simulink library "outp"  (R2021b)
(part 5 of 7)

  VPMM_ActiveDischargeReq_flg_Inproc : FVT_lib/outp/OverrideAndLimit  SystemSampleTime=-1  VariantActivationTime=update diagram  Latency=0  AutoFrameSizeCalculation=off
      link override Signal_Limit/_maxval: Value=KOUTP_ActiveDischargeReq_flg_maxval
      link override Signal_Limit/_minval: Value=KOUTP_ActiveDischargeReq_flg_minval
      link override Signal_Override/_ovrdflg: Value=KOUTP_ActiveDischargeReq_flg_ovrdflg
      link override Signal_Override/_ovrdval: Value=KOUTP_ActiveDischargeReq_flg_ovrdval
  VPMM_CtrlDrPwrStbA2_flg_Inproc : FVT_lib/outp/OverrideAndLimit  SystemSampleTime=-1  VariantActivationTime=update diagram  Latency=0  AutoFrameSizeCalculation=off
      link override Signal_Limit/_maxval: Value=KOUTP_CtrlDrPwrStbA2_flg_maxval
      link override Signal_Limit/_minval: Value=KOUTP_CtrlDrPwrStbA2_flg_minval
      link override Signal_Override/_ovrdflg: Value=KOUTP_CtrlDrPwrStbA2_flg_ovrdflg
      link override Signal_Override/_ovrdval: Value=KOUTP_CtrlDrPwrStbA2_flg_ovrdval
  VPMM_CtrlFrBMSCCUCIR_flg_Inproc : FVT_lib/outp/OverrideAndLimit  SystemSampleTime=-1  VariantActivationTime=update diagram  Latency=0  AutoFrameSizeCalculation=off
      link override Signal_Limit/_maxval: Value=KOUTP_CtrlFrBMSCCUCIR_flg_maxval
      link override Signal_Limit/_minval: Value=KOUTP_CtrlFrBMSCCUCIR_flg_minval
      link override Signal_Override/_ovrdflg: Value=KOUTP_CtrlFrBMSCCUCIR_flg_ovrdflg
      link override Signal_Override/_ovrdval: Value=KOUTP_CtrlFrBMSCCUCIR_flg_ovrdval
  VPMM_CtrlFrEDUINVERTER_flg_Inproc : FVT_lib/outp/OverrideAndLimit  SystemSampleTime=-1  VariantActivationTime=update diagram  Latency=0  AutoFrameSizeCalculation=off
      link override Signal_Limit/_maxval: Value=KOUTP_CtrlFrEDUINVERTER_flg_maxval
      link override Signal_Limit/_minval: Value=KOUTP_CtrlFrEDUINVERTER_flg_minval
      link override Signal_Override/_ovrdflg: Value=KOUTP_CtrlFrEDUINVERTER_flg_ovrdflg
      link override Signal_Override/_ovrdval: Value=KOUTP_CtrlFrEDUINVERTER_flg_ovrdval
  VPMM_CtrlFrPwrStbA1P_flg_Inproc : FVT_lib/outp/OverrideAndLimit  SystemSampleTime=-1  VariantActivationTime=update diagram  Latency=0  AutoFrameSizeCalculation=off
      link override Signal_Limit/_maxval: Value=KOUTP_CtrlFrPwrStbA1P_flg_maxval
      link override Signal_Limit/_minval: Value=KOUTP_CtrlFrPwrStbA1P_flg_minval
      link override Signal_Override/_ovrdflg: Value=KOUTP_CtrlFrPwrStbA1P_flg_ovrdflg
      link override Signal_Override/_ovrdval: Value=KOUTP_CtrlFrPwrStbA1P_flg_ovrdval
  VPMM_CtrlFrRC1_flg_Inproc : FVT_lib/outp/OverrideAndLimit  SystemSampleTime=-1  VariantActivationTime=update diagram  Latency=0  AutoFrameSizeCalculation=off
      link override Signal_Limit/_maxval: Value=KOUTP_CtrlFrRC1_flg_maxval
      link override Signal_Limit/_minval: Value=KOUTP_CtrlFrRC1_flg_minval
      link override Signal_Override/_ovrdflg: Value=KOUTP_CtrlFrRC1_flg_ovrdflg
      link override Signal_Override/_ovrdval: Value=KOUTP_CtrlFrRC1_flg_ovrdval
  VPMM_DCDCEnDem_enum_Inproc : FVT_lib/outp/OverrideAndLimit  SystemSampleTime=-1  VariantActivationTime=update diagram  Latency=0  AutoFrameSizeCalculation=off
      link override Signal_Limit/_maxval: Value=KOUTP_DCDCEnDem_enum_maxval
      link override Signal_Limit/_minval: Value=KOUTP_DCDCEnDem_enum_minval
      link override Signal_Override/_ovrdflg: Value=KOUTP_DCDCEnDem_enum_ovrdflg
      link override Signal_Override/_ovrdval: Value=KOUTP_DCDCEnDem_enum_ovrdval
  VPMM_DCDCEnaReq_flg_Inproc : FVT_lib/outp/OverrideAndLimit  SystemSampleTime=-1  VariantActivationTime=update diagram  Latency=0  AutoFrameSizeCalculation=off
      link override Signal_Limit/_maxval: Value=KOUTP_DCDCEnaReq_flg_maxval
      link override Signal_Limit/_minval: Value=KOUTP_DCDCEnaReq_flg_minval
      link override Signal_Override/_ovrdflg: Value=KOUTP_DCDCEnaReq_flg_ovrdflg
      link override Signal_Override/_ovrdval: Value=KOUTP_DCDCEnaReq_flg_ovrdval
  VPMM_DCDCRlyDem_enum_Inproc : FVT_lib/outp/OverrideAndLimit  SystemSampleTime=-1  VariantActivationTime=update diagram  Latency=0  AutoFrameSizeCalculation=off
      link override Signal_Limit/_maxval: Value=KOUTP_DCDCRlyDem_enum_maxval
      link override Signal_Limit/_minval: Value=KOUTP_DCDCRlyDem_enum_minval
      link override Signal_Override/_ovrdflg: Value=KOUTP_DCDCRlyDem_enum_ovrdflg
      link override Signal_Override/_ovrdval: Value=KOUTP_DCDCRlyDem_enum_ovrdval
  VPMM_DCDCVoltSetpoint_V_Inproc : FVT_lib/outp/OverrideAndLimit  SystemSampleTime=-1  VariantActivationTime=update diagram  Latency=0  AutoFrameSizeCalculation=off
      link override Signal_Limit/_maxval: Value=KOUTP_DCDCVoltSetpoint_V_maxval
      link override Signal_Limit/_minval: Value=KOUTP_DCDCVoltSetpoint_V_minval
      link override Signal_Override/_ovrdflg: Value=KOUTP_DCDCVoltSetpoint_V_ovrdflg
      link override Signal_Override/_ovrdval: Value=KOUTP_DCDCVoltSetpoint_V_ovrdval
  VPMM_DrSeatSta_enum_Inproc : FVT_lib/outp/OverrideAndLimit  SystemSampleTime=-1  VariantActivationTime=update diagram  Latency=0  AutoFrameSizeCalculation=off
      link override Signal_Limit/_maxval: Value=KOUTP_DrSeatSta_enum_maxval
      link override Signal_Limit/_minval: Value=KOUTP_DrSeatSta_enum_minval
      link override Signal_Override/_ovrdflg: Value=KOUTP_DrSeatSta_enum_ovrdflg
      link override Signal_Override/_ovrdval: Value=KOUTP_DrSeatSta_enum_ovrdval
  VPMM_DrivetrainSelect_enum_Inproc : FVT_lib/outp/OverrideAndLimit  SystemSampleTime=-1  VariantActivationTime=update diagram  Latency=0  AutoFrameSizeCalculation=off
      link override Signal_Limit/_maxval: Value=KOUTP_DrivetrainSelect_enum_maxval
      link override Signal_Limit/_minval: Value=KOUTP_DrivetrainSelect_enum_minval
      link override Signal_Override/_ovrdflg: Value=KOUTP_DrivetrainSelect_enum_ovrdflg
      link override Signal_Override/_ovrdval: Value=KOUTP_DrivetrainSelect_enum_ovrdval
  VPMM_EACRlyDem_enum_Inproc : FVT_lib/outp/OverrideAndLimit  SystemSampleTime=-1  VariantActivationTime=update diagram  Latency=0  AutoFrameSizeCalculation=off
      link override Signal_Limit/_maxval: Value=KOUTP_EACRlyDem_enum_maxval
      link override Signal_Limit/_minval: Value=KOUTP_EACRlyDem_enum_minval
      link override Signal_Override/_ovrdflg: Value=KOUTP_EACRlyDem_enum_ovrdflg
      link override Signal_Override/_ovrdval: Value=KOUTP_EACRlyDem_enum_ovrdval
  VPMM_EHPSRlyDem_enum_Inproc : FVT_lib/outp/OverrideAndLimit  SystemSampleTime=-1  VariantActivationTime=update diagram  Latency=0  AutoFrameSizeCalculation=off
      link override Signal_Limit/_maxval: Value=KOUTP_EHPSRlyDem_enum_maxval
      link override Signal_Limit/_minval: Value=KOUTP_EHPSRlyDem_enum_minval
      link override Signal_Override/_ovrdflg: Value=KOUTP_EHPSRlyDem_enum_ovrdflg
      link override Signal_Override/_ovrdval: Value=KOUTP_EHPSRlyDem_enum_ovrdval
  VPMM_EvccAplusPwrUpReq_flg_Inproc : FVT_lib/outp/OverrideAndLimit  SystemSampleTime=-1  VariantActivationTime=update diagram  Latency=0  AutoFrameSizeCalculation=off
      link override Signal_Limit/_maxval: Value=KOUTP_EvccAplusPwrUpReq_flg_maxval
      link override Signal_Limit/_minval: Value=KOUTP_EvccAplusPwrUpReq_flg_minval
      link override Signal_Override/_ovrdflg: Value=KOUTP_EvccAplusPwrUpReq_flg_ovrdflg
      link override Signal_Override/_ovrdval: Value=KOUTP_EvccAplusPwrUpReq_flg_ovrdval
  VPMM_FDADC12VDetAvg_mV_Inproc : FVT_lib/outp/OverrideAndLimit  SystemSampleTime=-1  VariantActivationTime=update diagram  Latency=0  AutoFrameSizeCalculation=off
      link override Signal_Limit/_maxval: Value=KOUTP_FDADC12VDetAvg_mV_maxval
      link override Signal_Limit/_minval: Value=KOUTP_FDADC12VDetAvg_mV_minval
      link override Signal_Override/_ovrdflg: Value=KOUTP_FDADC12VDetAvg_mV_ovrdflg
      link override Signal_Override/_ovrdval: Value=KOUTP_FDADC12VDetAvg_mV_ovrdval
  VPMM_FrMCUEnaReq_flg_Inproc : FVT_lib/outp/OverrideAndLimit  SystemSampleTime=-1  VariantActivationTime=update diagram  Latency=0  AutoFrameSizeCalculation=off
      link override Signal_Limit/_maxval: Value=KOUTP_FrMCUEnaReq_flg_maxval
      link override Signal_Limit/_minval: Value=KOUTP_FrMCUEnaReq_flg_minval
      link override Signal_Override/_ovrdflg: Value=KOUTP_FrMCUEnaReq_flg_ovrdflg
      link override Signal_Override/_ovrdval: Value=KOUTP_FrMCUEnaReq_flg_ovrdval
  VPMM_HVBatCnctReq_flg_Inproc : FVT_lib/outp/OverrideAndLimit  SystemSampleTime=-1  VariantActivationTime=update diagram  Latency=0  AutoFrameSizeCalculation=off
      link override Signal_Limit/_maxval: Value=KOUTP_HVBatCnctReq_flg_maxval
      link override Signal_Limit/_minval: Value=KOUTP_HVBatCnctReq_flg_minval
      link override Signal_Override/_ovrdflg: Value=KOUTP_HVBatCnctReq_flg_ovrdflg
      link override Signal_Override/_ovrdval: Value=KOUTP_HVBatCnctReq_flg_ovrdval
  VPMM_HVPwrSta_flg_Inproc : FVT_lib/outp/OverrideAndLimit  SystemSampleTime=-1  VariantActivationTime=update diagram  Latency=0  AutoFrameSizeCalculation=off
      link override Signal_Limit/_maxval: Value=KOUTP_HVPwrSta_flg_maxval
      link override Signal_Limit/_minval: Value=KOUTP_HVPwrSta_flg_minval
      link override Signal_Override/_ovrdflg: Value=KOUTP_HVPwrSta_flg_ovrdflg
      link override Signal_Override/_ovrdval: Value=KOUTP_HVPwrSta_flg_ovrdval
  VPMM_HVSysReadyToCharge_enum_Inproc : FVT_lib/outp/OverrideAndLimit  SystemSampleTime=-1  VariantActivationTime=update diagram  Latency=0  AutoFrameSizeCalculation=off
      link override Signal_Limit/_maxval: Value=KOUTP_HVSysReadyToCharge_enum_maxval
      link override Signal_Limit/_minval: Value=KOUTP_HVSysReadyToCharge_enum_minval
      link override Signal_Override/_ovrdflg: Value=KOUTP_HVSysReadyToCharge_enum_ovrdflg
      link override Signal_Override/_ovrdval: Value=KOUTP_HVSysReadyToCharge_enum_ovrdval
  VPMM_HWResetSta_enum_Inproc : FVT_lib/outp/OverrideAndLimit  SystemSampleTime=-1  VariantActivationTime=update diagram  Latency=0  AutoFrameSizeCalculation=off
      link override Signal_Limit/_maxval: Value=KOUTP_HWResetSta_enum_maxval
      link override Signal_Limit/_minval: Value=KOUTP_HWResetSta_enum_minval
      link override Signal_Override/_ovrdflg: Value=KOUTP_HWResetSta_enum_ovrdflg
      link override Signal_Override/_ovrdval: Value=KOUTP_HWResetSta_enum_ovrdval
  VPMM_IVIPwrStaONTOPopT_s_Inproc : FVT_lib/outp/OverrideAndLimit  SystemSampleTime=-1  VariantActivationTime=update diagram  Latency=0  AutoFrameSizeCalculation=off
      link override Signal_Limit/_maxval: Value=KOUTP_IVIPwrStaONTOPopT_s_maxval
      link override Signal_Limit/_minval: Value=KOUTP_IVIPwrStaONTOPopT_s_minval
      link override Signal_Override/_ovrdflg: Value=KOUTP_IVIPwrStaONTOPopT_s_ovrdflg
      link override Signal_Override/_ovrdval: Value=KOUTP_IVIPwrStaONTOPopT_s_ovrdval
  VPMM_LVBattChrgTimeCnt_s_Inproc : FVT_lib/outp/OverrideAndLimit  SystemSampleTime=-1  VariantActivationTime=update diagram  Latency=0  AutoFrameSizeCalculation=off
      link override Signal_Limit/_maxval: Value=KOUTP_LVBattChrgTimeCnt_s_maxval
      link override Signal_Limit/_minval: Value=KOUTP_LVBattChrgTimeCnt_s_minval
      link override Signal_Override/_ovrdflg: Value=KOUTP_LVBattChrgTimeCnt_s_ovrdflg
      link override Signal_Override/_ovrdval: Value=KOUTP_LVBattChrgTimeCnt_s_ovrdval
  VPMM_LVChrgHoldTtimer_s_Inproc : FVT_lib/outp/OverrideAndLimit  SystemSampleTime=-1  VariantActivationTime=update diagram  Latency=0  AutoFrameSizeCalculation=off
      link override Signal_Limit/_maxval: Value=KOUTP_LVChrgHoldTtimer_s_maxval
      link override Signal_Limit/_minval: Value=KOUTP_LVChrgHoldTtimer_s_minval
      link override Signal_Override/_ovrdflg: Value=KOUTP_LVChrgHoldTtimer_s_ovrdflg
      link override Signal_Override/_ovrdval: Value=KOUTP_LVChrgHoldTtimer_s_ovrdval
  VPMM_LVPwrSta_flg_Inproc : FVT_lib/outp/OverrideAndLimit  SystemSampleTime=-1  VariantActivationTime=update diagram  Latency=0  AutoFrameSizeCalculation=off
      link override Signal_Limit/_maxval: Value=KOUTP_LVPwrSta_flg_maxval
      link override Signal_Limit/_minval: Value=KOUTP_LVPwrSta_flg_minval
      link override Signal_Override/_ovrdflg: Value=KOUTP_LVPwrSta_flg_ovrdflg
      link override Signal_Override/_ovrdval: Value=KOUTP_LVPwrSta_flg_ovrdval
  VPMM_LVSilentChrgLv_enum_Inproc : FVT_lib/outp/OverrideAndLimit  SystemSampleTime=-1  VariantActivationTime=update diagram  Latency=0  AutoFrameSizeCalculation=off
      link override Signal_Limit/_maxval: Value=KOUTP_LVSilentChrgLv_enum_maxval
      link override Signal_Limit/_minval: Value=KOUTP_LVSilentChrgLv_enum_minval
      link override Signal_Override/_ovrdflg: Value=KOUTP_LVSilentChrgLv_enum_ovrdflg
      link override Signal_Override/_ovrdval: Value=KOUTP_LVSilentChrgLv_enum_ovrdval
  VPMM_LVSilentChrgReq_flg_Inproc : FVT_lib/outp/OverrideAndLimit  SystemSampleTime=-1  VariantActivationTime=update diagram  Latency=0  AutoFrameSizeCalculation=off
      link override Signal_Limit/_maxval: Value=KOUTP_LVSilentChrgReq_flg_maxval
      link override Signal_Limit/_minval: Value=KOUTP_LVSilentChrgReq_flg_minval
      link override Signal_Override/_ovrdflg: Value=KOUTP_LVSilentChrgReq_flg_ovrdflg
      link override Signal_Override/_ovrdval: Value=KOUTP_LVSilentChrgReq_flg_ovrdval
  VPMM_LVSilentChrgSta_enum_Inproc : FVT_lib/outp/OverrideAndLimit  SystemSampleTime=-1  VariantActivationTime=update diagram  Latency=0  AutoFrameSizeCalculation=off
      link override Signal_Limit/_maxval: Value=KOUTP_LVSilentChrgSta_enum_maxval
      link override Signal_Limit/_minval: Value=KOUTP_LVSilentChrgSta_enum_minval
      link override Signal_Override/_ovrdflg: Value=KOUTP_LVSilentChrgSta_enum_ovrdflg
      link override Signal_Override/_ovrdval: Value=KOUTP_LVSilentChrgSta_enum_ovrdval
  VPMM_LVSysErrPwrOutErr_flg_Inproc : FVT_lib/outp/OverrideAndLimit  SystemSampleTime=-1  VariantActivationTime=update diagram  Latency=0  AutoFrameSizeCalculation=off
      link override Signal_Limit/_maxval: Value=KOUTP_LVSysErrPwrOutErr_flg_maxval
      link override Signal_Limit/_minval: Value=KOUTP_LVSysErrPwrOutErr_flg_minval
      link override Signal_Override/_ovrdflg: Value=KOUTP_LVSysErrPwrOutErr_flg_ovrdflg
      link override Signal_Override/_ovrdval: Value=KOUTP_LVSysErrPwrOutErr_flg_ovrdval
  VPMM_LowSOCWarn_enum_Inproc : FVT_lib/outp/OverrideAndLimit  SystemSampleTime=-1  VariantActivationTime=update diagram  Latency=0  AutoFrameSizeCalculation=off
      link override Signal_Limit/_maxval: Value=KOUTP_LowSOCWarn_enum_maxval
      link override Signal_Limit/_minval: Value=KOUTP_LowSOCWarn_enum_minval
      link override Signal_Override/_ovrdflg: Value=KOUTP_LowSOCWarn_enum_ovrdflg
      link override Signal_Override/_ovrdval: Value=KOUTP_LowSOCWarn_enum_ovrdval
  VPMM_PMMAllowECUSleep_flg_Inproc : FVT_lib/outp/OverrideAndLimit  SystemSampleTime=-1  VariantActivationTime=update diagram  Latency=0  AutoFrameSizeCalculation=off
      link override Signal_Limit/_maxval: Value=KOUTP_PMMAllowECUSleep_flg_maxval
      link override Signal_Limit/_minval: Value=KOUTP_PMMAllowECUSleep_flg_minval
      link override Signal_Override/_ovrdflg: Value=KOUTP_PMMAllowECUSleep_flg_ovrdflg
      link override Signal_Override/_ovrdval: Value=KOUTP_PMMAllowECUSleep_flg_ovrdval
  VPMM_PowerDownFault_enum_Inproc : FVT_lib/outp/OverrideAndLimit  SystemSampleTime=-1  VariantActivationTime=update diagram  Latency=0  AutoFrameSizeCalculation=off
      link override Signal_Limit/_maxval: Value=KOUTP_PowerDownFault_enum_maxval
      link override Signal_Limit/_minval: Value=KOUTP_PowerDownFault_enum_minval
      link override Signal_Override/_ovrdflg: Value=KOUTP_PowerDownFault_enum_ovrdflg
      link override Signal_Override/_ovrdval: Value=KOUTP_PowerDownFault_enum_ovrdval
  VPMM_PowerDownState_enum_Inproc : FVT_lib/outp/OverrideAndLimit  SystemSampleTime=-1  VariantActivationTime=update diagram  Latency=0  AutoFrameSizeCalculation=off
      link override Signal_Limit/_maxval: Value=KOUTP_PowerDownState_enum_maxval
      link override Signal_Limit/_minval: Value=KOUTP_PowerDownState_enum_minval
      link override Signal_Override/_ovrdflg: Value=KOUTP_PowerDownState_enum_ovrdflg
      link override Signal_Override/_ovrdval: Value=KOUTP_PowerDownState_enum_ovrdval
  VPMM_PowerSta_enum_Inproc : FVT_lib/outp/OverrideAndLimit  SystemSampleTime=-1  VariantActivationTime=update diagram  Latency=0  AutoFrameSizeCalculation=off
      link override Signal_Limit/_maxval: Value=KOUTP_PowerSta_enum_maxval
      link override Signal_Limit/_minval: Value=KOUTP_PowerSta_enum_minval
      link override Signal_Override/_ovrdflg: Value=KOUTP_PowerSta_enum_ovrdflg
      link override Signal_Override/_ovrdval: Value=KOUTP_PowerSta_enum_ovrdval
  VPMM_PowerUpFault_enum_Inproc : FVT_lib/outp/OverrideAndLimit  SystemSampleTime=-1  VariantActivationTime=update diagram  Latency=0  AutoFrameSizeCalculation=off
      link override Signal_Limit/_maxval: Value=KOUTP_PowerUpFault_enum_maxval
      link override Signal_Limit/_minval: Value=KOUTP_PowerUpFault_enum_minval
      link override Signal_Override/_ovrdflg: Value=KOUTP_PowerUpFault_enum_ovrdflg
      link override Signal_Override/_ovrdval: Value=KOUTP_PowerUpFault_enum_ovrdval
  VPMM_PowerUpState_enum_Inproc : FVT_lib/outp/OverrideAndLimit  SystemSampleTime=-1  VariantActivationTime=update diagram  Latency=0  AutoFrameSizeCalculation=off
      link override Signal_Limit/_maxval: Value=KOUTP_PowerUpState_enum_maxval
      link override Signal_Limit/_minval: Value=KOUTP_PowerUpState_enum_minval
      link override Signal_Override/_ovrdflg: Value=KOUTP_PowerUpState_enum_ovrdflg
      link override Signal_Override/_ovrdval: Value=KOUTP_PowerUpState_enum_ovrdval
  VPMM_PwrDownReq_enum_Inproc : FVT_lib/outp/OverrideAndLimit  SystemSampleTime=-1  VariantActivationTime=update diagram  Latency=0  AutoFrameSizeCalculation=off
      link override Signal_Limit/_maxval: Value=KOUTP_PwrDownReq_enum_maxval
      link override Signal_Limit/_minval: Value=KOUTP_PwrDownReq_enum_minval
      link override Signal_Override/_ovrdflg: Value=KOUTP_PwrDownReq_enum_ovrdflg
      link override Signal_Override/_ovrdval: Value=KOUTP_PwrDownReq_enum_ovrdval
  VPMM_PwrStaConstraint_enum_Inproc : FVT_lib/outp/OverrideAndLimit  SystemSampleTime=-1  VariantActivationTime=update diagram  Latency=0  AutoFrameSizeCalculation=off
      link override Signal_Limit/_maxval: Value=KOUTP_PwrStaConstraint_enum_maxval
      link override Signal_Limit/_minval: Value=KOUTP_PwrStaConstraint_enum_minval
      link override Signal_Override/_ovrdflg: Value=KOUTP_PwrStaConstraint_enum_ovrdflg
      link override Signal_Override/_ovrdval: Value=KOUTP_PwrStaConstraint_enum_ovrdval
  VPMM_PwrStaONTOPopReq_flg_Inproc : FVT_lib/outp/OverrideAndLimit  SystemSampleTime=-1  VariantActivationTime=update diagram  Latency=0  AutoFrameSizeCalculation=off
      link override Signal_Limit/_maxval: Value=KOUTP_PwrStaONTOPopReq_flg_maxval
      link override Signal_Limit/_minval: Value=KOUTP_PwrStaONTOPopReq_flg_minval
      link override Signal_Override/_ovrdflg: Value=KOUTP_PwrStaONTOPopReq_flg_ovrdflg
      link override Signal_Override/_ovrdval: Value=KOUTP_PwrStaONTOPopReq_flg_ovrdval
  VPMM_PwrStaSelect_enum_Inproc : FVT_lib/outp/OverrideAndLimit  SystemSampleTime=-1  VariantActivationTime=update diagram  Latency=0  AutoFrameSizeCalculation=off
      link override Signal_Limit/_maxval: Value=KOUTP_PwrStaSelect_enum_maxval
      link override Signal_Limit/_minval: Value=KOUTP_PwrStaSelect_enum_minval
      link override Signal_Override/_ovrdflg: Value=KOUTP_PwrStaSelect_enum_ovrdflg
      link override Signal_Override/_ovrdval: Value=KOUTP_PwrStaSelect_enum_ovrdval
  VPMM_PwrStaTOSta_enum_Inproc : FVT_lib/outp/OverrideAndLimit  SystemSampleTime=-1  VariantActivationTime=update diagram  Latency=0  AutoFrameSizeCalculation=off
      link override Signal_Limit/_maxval: Value=KOUTP_PwrStaTOSta_enum_maxval
      link override Signal_Limit/_minval: Value=KOUTP_PwrStaTOSta_enum_minval
      link override Signal_Override/_ovrdflg: Value=KOUTP_PwrStaTOSta_enum_ovrdflg
      link override Signal_Override/_ovrdval: Value=KOUTP_PwrStaTOSta_enum_ovrdval
  VPMM_PwrUpReq_enum_Inproc : FVT_lib/outp/OverrideAndLimit  SystemSampleTime=-1  VariantActivationTime=update diagram  Latency=0  AutoFrameSizeCalculation=off
      link override Signal_Limit/_maxval: Value=KOUTP_PwrUpReq_enum_maxval
      link override Signal_Limit/_minval: Value=KOUTP_PwrUpReq_enum_minval
      link override Signal_Override/_ovrdflg: Value=KOUTP_PwrUpReq_enum_ovrdflg
      link override Signal_Override/_ovrdval: Value=KOUTP_PwrUpReq_enum_ovrdval
  VPMM_ReVehThdChkSta_enum_Inproc : FVT_lib/outp/OverrideAndLimit  SystemSampleTime=-1  VariantActivationTime=update diagram  Latency=0  AutoFrameSizeCalculation=off
      link override Signal_Limit/_maxval: Value=KOUTP_ReVehThdChkSta_enum_maxval
      link override Signal_Limit/_minval: Value=KOUTP_ReVehThdChkSta_enum_minval
      link override Signal_Override/_ovrdflg: Value=KOUTP_ReVehThdChkSta_enum_ovrdflg
      link override Signal_Override/_ovrdval: Value=KOUTP_ReVehThdChkSta_enum_ovrdval
  VPMM_RrMCUEnaReq_flg_Inproc : FVT_lib/outp/OverrideAndLimit  SystemSampleTime=-1  VariantActivationTime=update diagram  Latency=0  AutoFrameSizeCalculation=off
      link override Signal_Limit/_maxval: Value=KOUTP_RrMCUEnaReq_flg_maxval
      link override Signal_Limit/_minval: Value=KOUTP_RrMCUEnaReq_flg_minval
      link override Signal_Override/_ovrdflg: Value=KOUTP_RrMCUEnaReq_flg_ovrdflg
      link override Signal_Override/_ovrdval: Value=KOUTP_RrMCUEnaReq_flg_ovrdval
  VPMM_SilentChkAllowSleep_flg_Inproc : FVT_lib/outp/OverrideAndLimit  SystemSampleTime=-1  VariantActivationTime=update diagram  Latency=0  AutoFrameSizeCalculation=off
      link override Signal_Limit/_maxval: Value=KOUTP_SilentChkAllowSleep_flg_maxval
      link override Signal_Limit/_minval: Value=KOUTP_SilentChkAllowSleep_flg_minval
      link override Signal_Override/_ovrdflg: Value=KOUTP_SilentChkAllowSleep_flg_ovrdflg
      link override Signal_Override/_ovrdval: Value=KOUTP_SilentChkAllowSleep_flg_ovrdval
  VPMM_SysPowerMode_enum_Inproc : FVT_lib/outp/OverrideAndLimit  SystemSampleTime=-1  VariantActivationTime=update diagram  Latency=0  AutoFrameSizeCalculation=off
      link override Signal_Limit/_maxval: Value=KOUTP_SysPowerMode_enum_maxval
      link override Signal_Limit/_minval: Value=KOUTP_SysPowerMode_enum_minval
      link override Signal_Override/_ovrdflg: Value=KOUTP_SysPowerMode_enum_ovrdflg
      link override Signal_Override/_ovrdval: Value=KOUTP_SysPowerMode_enum_ovrdval
  VPMM_TCountSta_enum_Inproc : FVT_lib/outp/OverrideAndLimit  SystemSampleTime=-1  VariantActivationTime=update diagram  Latency=0  AutoFrameSizeCalculation=off
      link override Signal_Limit/_maxval: Value=KOUTP_TCountSta_enum_maxval
      link override Signal_Limit/_minval: Value=KOUTP_TCountSta_enum_minval
      link override Signal_Override/_ovrdflg: Value=KOUTP_TCountSta_enum_ovrdflg
      link override Signal_Override/_ovrdval: Value=KOUTP_TCountSta_enum_ovrdval
  VPMM_TimerAllowSleep_flg_Inproc : FVT_lib/outp/OverrideAndLimit  SystemSampleTime=-1  VariantActivationTime=update diagram  Latency=0  AutoFrameSizeCalculation=off
      link override Signal_Limit/_maxval: Value=KOUTP_TimerAllowSleep_flg_maxval
      link override Signal_Limit/_minval: Value=KOUTP_TimerAllowSleep_flg_minval
      link override Signal_Override/_ovrdflg: Value=KOUTP_TimerAllowSleep_flg_ovrdflg
      link override Signal_Override/_ovrdval: Value=KOUTP_TimerAllowSleep_flg_ovrdval
  VSCP_ABSActive_flg_Inproc : FVT_lib/outp/OverrideAndLimit  SystemSampleTime=-1  VariantActivationTime=update diagram  Latency=0  AutoFrameSizeCalculation=off
      link override Signal_Limit/_maxval: Value=KOUTP_ABSActive_flg_maxval
      link override Signal_Limit/_minval: Value=KOUTP_ABSActive_flg_minval
      link override Signal_Override/_ovrdflg: Value=KOUTP_ABSActive_flg_ovrdflg
      link override Signal_Override/_ovrdval: Value=KOUTP_ABSActive_flg_ovrdval
  VSCP_ABSFailed_flg_Inproc : FVT_lib/outp/OverrideAndLimit  SystemSampleTime=-1  VariantActivationTime=update diagram  Latency=0  AutoFrameSizeCalculation=off
      link override Signal_Limit/_maxval: Value=KOUTP_ABSFailed_flg_maxval
      link override Signal_Limit/_minval: Value=KOUTP_ABSFailed_flg_minval
      link override Signal_Override/_ovrdflg: Value=KOUTP_ABSFailed_flg_ovrdflg
      link override Signal_Override/_ovrdval: Value=KOUTP_ABSFailed_flg_ovrdval
  VSCP_ABSWnlmpSta_flg_Inproc : FVT_lib/outp/OverrideAndLimit  SystemSampleTime=-1  VariantActivationTime=update diagram  Latency=0  AutoFrameSizeCalculation=off
      link override Signal_Limit/_maxval: Value=KOUTP_ABSWnlmpSta_flg_maxval
      link override Signal_Limit/_minval: Value=KOUTP_ABSWnlmpSta_flg_minval
      link override Signal_Override/_ovrdflg: Value=KOUTP_ABSWnlmpSta_flg_ovrdflg
      link override Signal_Override/_ovrdval: Value=KOUTP_ABSWnlmpSta_flg_ovrdval
  VSCP_AmberWnlmpSta_flg_Inproc : FVT_lib/outp/OverrideAndLimit  SystemSampleTime=-1  VariantActivationTime=update diagram  Latency=0  AutoFrameSizeCalculation=off
      link override Signal_Limit/_maxval: Value=KOUTP_AmberWnlmpSta_flg_maxval
      link override Signal_Limit/_minval: Value=KOUTP_AmberWnlmpSta_flg_minval
      link override Signal_Override/_ovrdflg: Value=KOUTP_AmberWnlmpSta_flg_ovrdflg
      link override Signal_Override/_ovrdval: Value=KOUTP_AmberWnlmpSta_flg_ovrdval
  VSCP_BrkPedalPos_pct_Inproc : FVT_lib/outp/OverrideAndLimit  SystemSampleTime=-1  VariantActivationTime=update diagram  Latency=0  AutoFrameSizeCalculation=off
      link override Signal_Limit/_maxval: Value=KOUTP_BrkPedalPos_pct_maxval
      link override Signal_Limit/_minval: Value=KOUTP_BrkPedalPos_pct_minval
      link override Signal_Override/_ovrdflg: Value=KOUTP_BrkPedalPos_pct_ovrdflg
      link override Signal_Override/_ovrdval: Value=KOUTP_BrkPedalPos_pct_ovrdval
  VSCP_CFGEM1BAMPGN_raw_Inproc : FVT_lib/outp/OverrideAndLimit  SystemSampleTime=-1  VariantActivationTime=update diagram  Latency=0  AutoFrameSizeCalculation=off
      link override Signal_Limit/_maxval: Value=KOUTP_CFGEM1BAMPGN_raw_maxval
      link override Signal_Limit/_minval: Value=KOUTP_CFGEM1BAMPGN_raw_minval
      link override Signal_Override/_ovrdflg: Value=KOUTP_CFGEM1BAMPGN_raw_ovrdflg
      link override Signal_Override/_ovrdval: Value=KOUTP_CFGEM1BAMPGN_raw_ovrdval
  VSCP_CFGEM1BAMRsv_raw_Inproc : FVT_lib/outp/OverrideAndLimit  SystemSampleTime=-1  VariantActivationTime=update diagram  Latency=0  AutoFrameSizeCalculation=off
      link override Signal_Limit/_maxval: Value=KOUTP_CFGEM1BAMRsv_raw_maxval
      link override Signal_Limit/_minval: Value=KOUTP_CFGEM1BAMRsv_raw_minval
      link override Signal_Override/_ovrdflg: Value=KOUTP_CFGEM1BAMRsv_raw_ovrdflg
      link override Signal_Override/_ovrdval: Value=KOUTP_CFGEM1BAMRsv_raw_ovrdval
  VSCP_CFGEM1BAMTNum_raw_Inproc : FVT_lib/outp/OverrideAndLimit  SystemSampleTime=-1  VariantActivationTime=update diagram  Latency=0  AutoFrameSizeCalculation=off
      link override Signal_Limit/_maxval: Value=KOUTP_CFGEM1BAMTNum_raw_maxval
      link override Signal_Limit/_minval: Value=KOUTP_CFGEM1BAMTNum_raw_minval
      link override Signal_Override/_ovrdflg: Value=KOUTP_CFGEM1BAMTNum_raw_ovrdflg
      link override Signal_Override/_ovrdval: Value=KOUTP_CFGEM1BAMTNum_raw_ovrdval
  VSCP_CFGEM1BAMTSize_raw_Inproc : FVT_lib/outp/OverrideAndLimit  SystemSampleTime=-1  VariantActivationTime=update diagram  Latency=0  AutoFrameSizeCalculation=off
      link override Signal_Limit/_maxval: Value=KOUTP_CFGEM1BAMTSize_raw_maxval
      link override Signal_Limit/_minval: Value=KOUTP_CFGEM1BAMTSize_raw_minval
      link override Signal_Override/_ovrdflg: Value=KOUTP_CFGEM1BAMTSize_raw_ovrdflg
      link override Signal_Override/_ovrdval: Value=KOUTP_CFGEM1BAMTSize_raw_ovrdval
  VSCP_CFGEM1Ctrl_raw_Inproc : FVT_lib/outp/OverrideAndLimit  SystemSampleTime=-1  VariantActivationTime=update diagram  Latency=0  AutoFrameSizeCalculation=off
      link override Signal_Limit/_maxval: Value=KOUTP_CFGEM1Ctrl_raw_maxval
      link override Signal_Limit/_minval: Value=KOUTP_CFGEM1Ctrl_raw_minval
      link override Signal_Override/_ovrdflg: Value=KOUTP_CFGEM1Ctrl_raw_ovrdflg
      link override Signal_Override/_ovrdval: Value=KOUTP_CFGEM1Ctrl_raw_ovrdval
  VSCP_DTbyte0_raw_Inproc : FVT_lib/outp/OverrideAndLimit  SystemSampleTime=-1  VariantActivationTime=update diagram  Latency=0  AutoFrameSizeCalculation=off
      link override Signal_Limit/_maxval: Value=KOUTP_DTbyte0_raw_maxval
      link override Signal_Limit/_minval: Value=KOUTP_DTbyte0_raw_minval
      link override Signal_Override/_ovrdflg: Value=KOUTP_DTbyte0_raw_ovrdflg
      link override Signal_Override/_ovrdval: Value=KOUTP_DTbyte0_raw_ovrdval
  VSCP_DTbyte1_raw_Inproc : FVT_lib/outp/OverrideAndLimit  SystemSampleTime=-1  VariantActivationTime=update diagram  Latency=0  AutoFrameSizeCalculation=off
      link override Signal_Limit/_maxval: Value=KOUTP_DTbyte1_raw_maxval
      link override Signal_Limit/_minval: Value=KOUTP_DTbyte1_raw_minval
      link override Signal_Override/_ovrdflg: Value=KOUTP_DTbyte1_raw_ovrdflg
      link override Signal_Override/_ovrdval: Value=KOUTP_DTbyte1_raw_ovrdval
  VSCP_DTbyte2_raw_Inproc : FVT_lib/outp/OverrideAndLimit  SystemSampleTime=-1  VariantActivationTime=update diagram  Latency=0  AutoFrameSizeCalculation=off
      link override Signal_Limit/_maxval: Value=KOUTP_DTbyte2_raw_maxval
      link override Signal_Limit/_minval: Value=KOUTP_DTbyte2_raw_minval
      link override Signal_Override/_ovrdflg: Value=KOUTP_DTbyte2_raw_ovrdflg
      link override Signal_Override/_ovrdval: Value=KOUTP_DTbyte2_raw_ovrdval
  VSCP_DTbyte3_raw_Inproc : FVT_lib/outp/OverrideAndLimit  SystemSampleTime=-1  VariantActivationTime=update diagram  Latency=0  AutoFrameSizeCalculation=off
      link override Signal_Limit/_maxval: Value=KOUTP_DTbyte3_raw_maxval
      link override Signal_Limit/_minval: Value=KOUTP_DTbyte3_raw_minval
      link override Signal_Override/_ovrdflg: Value=KOUTP_DTbyte3_raw_ovrdflg
      link override Signal_Override/_ovrdval: Value=KOUTP_DTbyte3_raw_ovrdval
  VSCP_DTbyte4_raw_Inproc : FVT_lib/outp/OverrideAndLimit  SystemSampleTime=-1  VariantActivationTime=update diagram  Latency=0  AutoFrameSizeCalculation=off
      link override Signal_Limit/_maxval: Value=KOUTP_DTbyte4_raw_maxval
      link override Signal_Limit/_minval: Value=KOUTP_DTbyte4_raw_minval
      link override Signal_Override/_ovrdflg: Value=KOUTP_DTbyte4_raw_ovrdflg
      link override Signal_Override/_ovrdval: Value=KOUTP_DTbyte4_raw_ovrdval
  VSCP_DTbyte5_raw_Inproc : FVT_lib/outp/OverrideAndLimit  SystemSampleTime=-1  VariantActivationTime=update diagram  Latency=0  AutoFrameSizeCalculation=off
      link override Signal_Limit/_maxval: Value=KOUTP_DTbyte5_raw_maxval
      link override Signal_Limit/_minval: Value=KOUTP_DTbyte5_raw_minval
      link override Signal_Override/_ovrdflg: Value=KOUTP_DTbyte5_raw_ovrdflg
      link override Signal_Override/_ovrdval: Value=KOUTP_DTbyte5_raw_ovrdval
  VSCP_DTbyte6_raw_Inproc : FVT_lib/outp/OverrideAndLimit  SystemSampleTime=-1  VariantActivationTime=update diagram  Latency=0  AutoFrameSizeCalculation=off
      link override Signal_Limit/_maxval: Value=KOUTP_DTbyte6_raw_maxval
      link override Signal_Limit/_minval: Value=KOUTP_DTbyte6_raw_minval
      link override Signal_Override/_ovrdflg: Value=KOUTP_DTbyte6_raw_ovrdflg
      link override Signal_Override/_ovrdval: Value=KOUTP_DTbyte6_raw_ovrdval
  VSCP_DTbyte7_raw_Inproc : FVT_lib/outp/OverrideAndLimit  SystemSampleTime=-1  VariantActivationTime=update diagram  Latency=0  AutoFrameSizeCalculation=off
      link override Signal_Limit/_maxval: Value=KOUTP_DTbyte7_raw_maxval
      link override Signal_Limit/_minval: Value=KOUTP_DTbyte7_raw_minval
      link override Signal_Override/_ovrdflg: Value=KOUTP_DTbyte7_raw_ovrdflg
      link override Signal_Override/_ovrdval: Value=KOUTP_DTbyte7_raw_ovrdval
  VSCP_HSAActive_flg_Inproc : FVT_lib/outp/OverrideAndLimit  SystemSampleTime=-1  VariantActivationTime=update diagram  Latency=0  AutoFrameSizeCalculation=off
      link override Signal_Limit/_maxval: Value=KOUTP_HSAActive_flg_maxval
      link override Signal_Limit/_minval: Value=KOUTP_HSAActive_flg_minval
      link override Signal_Override/_ovrdflg: Value=KOUTP_HSAActive_flg_ovrdflg
      link override Signal_Override/_ovrdval: Value=KOUTP_HSAActive_flg_ovrdval
  VSCP_HSAFailed_flg_Inproc : FVT_lib/outp/OverrideAndLimit  SystemSampleTime=-1  VariantActivationTime=update diagram  Latency=0  AutoFrameSizeCalculation=off
      link override Signal_Limit/_maxval: Value=KOUTP_HSAFailed_flg_maxval
      link override Signal_Limit/_minval: Value=KOUTP_HSAFailed_flg_minval
      link override Signal_Override/_ovrdflg: Value=KOUTP_HSAFailed_flg_ovrdflg
      link override Signal_Override/_ovrdval: Value=KOUTP_HSAFailed_flg_ovrdval
  VSCP_MeterIndVehSpeed_kph_Inproc : FVT_lib/outp/OverrideAndLimit  SystemSampleTime=-1  VariantActivationTime=update diagram  Latency=0  AutoFrameSizeCalculation=off
      link override Signal_Limit/_maxval: Value=KOUTP_MeterIndVehSpeed_kph_maxval
      link override Signal_Limit/_minval: Value=KOUTP_MeterIndVehSpeed_kph_minval
      link override Signal_Override/_ovrdflg: Value=KOUTP_MeterIndVehSpeed_kph_ovrdflg
      link override Signal_Override/_ovrdval: Value=KOUTP_MeterIndVehSpeed_kph_ovrdval
  VSCP_OpenStatusOfDoor1_enum_Inproc : FVT_lib/outp/OverrideAndLimit  SystemSampleTime=-1  VariantActivationTime=update diagram  Latency=0  AutoFrameSizeCalculation=off
      link override Signal_Limit/_maxval: Value=KOUTP_OpenStatusOfDoor1_enum_maxval
      link override Signal_Limit/_minval: Value=KOUTP_OpenStatusOfDoor1_enum_minval
      link override Signal_Override/_ovrdflg: Value=KOUTP_OpenStatusOfDoor1_enum_ovrdflg
      link override Signal_Override/_ovrdval: Value=KOUTP_OpenStatusOfDoor1_enum_ovrdval
  VSCP_OpenStatusOfDoor2_enum_Inproc : FVT_lib/outp/OverrideAndLimit  SystemSampleTime=-1  VariantActivationTime=update diagram  Latency=0  AutoFrameSizeCalculation=off
      link override Signal_Limit/_maxval: Value=KOUTP_OpenStatusOfDoor2_enum_maxval
      link override Signal_Limit/_minval: Value=KOUTP_OpenStatusOfDoor2_enum_minval
      link override Signal_Override/_ovrdflg: Value=KOUTP_OpenStatusOfDoor2_enum_ovrdflg
      link override Signal_Override/_ovrdval: Value=KOUTP_OpenStatusOfDoor2_enum_ovrdval
  VSCP_RedWnlmpSta_flg_Inproc : FVT_lib/outp/OverrideAndLimit  SystemSampleTime=-1  VariantActivationTime=update diagram  Latency=0  AutoFrameSizeCalculation=off
      link override Signal_Limit/_maxval: Value=KOUTP_RedWnlmpSta_flg_maxval
      link override Signal_Limit/_minval: Value=KOUTP_RedWnlmpSta_flg_minval
      link override Signal_Override/_ovrdflg: Value=KOUTP_RedWnlmpSta_flg_ovrdflg
      link override Signal_Override/_ovrdval: Value=KOUTP_RedWnlmpSta_flg_ovrdval
  VSCP_SCPBrkSwSta_flg_Inproc : FVT_lib/outp/OverrideAndLimit  SystemSampleTime=-1  VariantActivationTime=update diagram  Latency=0  AutoFrameSizeCalculation=off
      link override Signal_Limit/_maxval: Value=KOUTP_SCPBrkSwSta_flg_maxval
      link override Signal_Limit/_minval: Value=KOUTP_SCPBrkSwSta_flg_minval
      link override Signal_Override/_ovrdflg: Value=KOUTP_SCPBrkSwSta_flg_ovrdflg
      link override Signal_Override/_ovrdval: Value=KOUTP_SCPBrkSwSta_flg_ovrdval
  VSCP_SeatBeltSwitch_enum_Inproc : FVT_lib/outp/OverrideAndLimit  SystemSampleTime=-1  VariantActivationTime=update diagram  Latency=0  AutoFrameSizeCalculation=off
      link override Signal_Limit/_maxval: Value=KOUTP_SeatBeltSwitch_enum_maxval
      link override Signal_Limit/_minval: Value=KOUTP_SeatBeltSwitch_enum_minval
      link override Signal_Override/_ovrdflg: Value=KOUTP_SeatBeltSwitch_enum_ovrdflg
      link override Signal_Override/_ovrdval: Value=KOUTP_SeatBeltSwitch_enum_ovrdval
  VSCP_Vehspeed_kph_Inproc : FVT_lib/outp/OverrideAndLimit  SystemSampleTime=-1  VariantActivationTime=update diagram  Latency=0  AutoFrameSizeCalculation=off
      link override Signal_Limit/_maxval: Value=KOUTP_Vehspeed_kph_maxval
      link override Signal_Limit/_minval: Value=KOUTP_Vehspeed_kph_minval
      link override Signal_Override/_ovrdflg: Value=KOUTP_Vehspeed_kph_ovrdflg
      link override Signal_Override/_ovrdval: Value=KOUTP_Vehspeed_kph_ovrdval
  VSCP_triggerBAM_flg_Inproc : FVT_lib/outp/OverrideAndLimit  SystemSampleTime=-1  VariantActivationTime=update diagram  Latency=0  AutoFrameSizeCalculation=off
      link override Signal_Limit/_maxval: Value=KOUTP_triggerBAM_flg_maxval
      link override Signal_Limit/_minval: Value=KOUTP_triggerBAM_flg_minval
      link override Signal_Override/_ovrdflg: Value=KOUTP_triggerBAM_flg_ovrdflg
      link override Signal_Override/_ovrdval: Value=KOUTP_triggerBAM_flg_ovrdval
  VSCP_triggerDT_flg_Inproc : FVT_lib/outp/OverrideAndLimit  SystemSampleTime=-1  VariantActivationTime=update diagram  Latency=0  AutoFrameSizeCalculation=off
      link override Signal_Limit/_maxval: Value=KOUTP_triggerDT_flg_maxval
      link override Signal_Limit/_minval: Value=KOUTP_triggerDT_flg_minval
      link override Signal_Override/_ovrdflg: Value=KOUTP_triggerDT_flg_ovrdflg
      link override Signal_Override/_ovrdval: Value=KOUTP_triggerDT_flg_ovrdval
  VSYS_AcoreRebootCmdACK_flg_Inproc : FVT_lib/outp/OverrideAndLimit  SystemSampleTime=-1  VariantActivationTime=update diagram  Latency=0  AutoFrameSizeCalculation=off
      link override Signal_Limit/_maxval: Value=KOUTP_AcoreRebootCmdACK_flg_maxval
      link override Signal_Limit/_minval: Value=KOUTP_AcoreRebootCmdACK_flg_minval
      link override Signal_Override/_ovrdflg: Value=KOUTP_AcoreRebootCmdACK_flg_ovrdflg
      link override Signal_Override/_ovrdval: Value=KOUTP_AcoreRebootCmdACK_flg_ovrdval
  VSYS_CarModel1_cnt_Inproc : FVT_lib/outp/OverrideAndLimit  SystemSampleTime=-1  VariantActivationTime=update diagram  Latency=0  AutoFrameSizeCalculation=off
      link override Signal_Limit/_maxval: Value=KOUTP_CarModel1_cnt_maxval
      link override Signal_Limit/_minval: Value=KOUTP_CarModel1_cnt_minval
      link override Signal_Override/_ovrdflg: Value=KOUTP_CarModel1_cnt_ovrdflg
      link override Signal_Override/_ovrdval: Value=KOUTP_CarModel1_cnt_ovrdval
  VSYS_CarModel2_cnt_Inproc : FVT_lib/outp/OverrideAndLimit  SystemSampleTime=-1  VariantActivationTime=update diagram  Latency=0  AutoFrameSizeCalculation=off
      link override Signal_Limit/_maxval: Value=KOUTP_CarModel2_cnt_maxval
      link override Signal_Limit/_minval: Value=KOUTP_CarModel2_cnt_minval
      link override Signal_Override/_ovrdflg: Value=KOUTP_CarModel2_cnt_ovrdflg
      link override Signal_Override/_ovrdval: Value=KOUTP_CarModel2_cnt_ovrdval
  VSYS_CarModel3_cnt_Inproc : FVT_lib/outp/OverrideAndLimit  SystemSampleTime=-1  VariantActivationTime=update diagram  Latency=0  AutoFrameSizeCalculation=off
      link override Signal_Limit/_maxval: Value=KOUTP_CarModel3_cnt_maxval
      link override Signal_Limit/_minval: Value=KOUTP_CarModel3_cnt_minval
      link override Signal_Override/_ovrdflg: Value=KOUTP_CarModel3_cnt_ovrdflg
      link override Signal_Override/_ovrdval: Value=KOUTP_CarModel3_cnt_ovrdval
  VSYS_Change1_cnt_Inproc : FVT_lib/outp/OverrideAndLimit  SystemSampleTime=-1  VariantActivationTime=update diagram  Latency=0  AutoFrameSizeCalculation=off
      link override Signal_Limit/_maxval: Value=KOUTP_Change1_cnt_maxval
      link override Signal_Limit/_minval: Value=KOUTP_Change1_cnt_minval
      link override Signal_Override/_ovrdflg: Value=KOUTP_Change1_cnt_ovrdflg
      link override Signal_Override/_ovrdval: Value=KOUTP_Change1_cnt_ovrdval
  VSYS_Change2_cnt_Inproc : FVT_lib/outp/OverrideAndLimit  SystemSampleTime=-1  VariantActivationTime=update diagram  Latency=0  AutoFrameSizeCalculation=off
      link override Signal_Limit/_maxval: Value=KOUTP_Change2_cnt_maxval
      link override Signal_Limit/_minval: Value=KOUTP_Change2_cnt_minval
      link override Signal_Override/_ovrdflg: Value=KOUTP_Change2_cnt_ovrdflg
      link override Signal_Override/_ovrdval: Value=KOUTP_Change2_cnt_ovrdval
  VSYS_Country1_cnt_Inproc : FVT_lib/outp/OverrideAndLimit  SystemSampleTime=-1  VariantActivationTime=update diagram  Latency=0  AutoFrameSizeCalculation=off
      link override Signal_Limit/_maxval: Value=KOUTP_Country1_cnt_maxval
      link override Signal_Limit/_minval: Value=KOUTP_Country1_cnt_minval
      link override Signal_Override/_ovrdflg: Value=KOUTP_Country1_cnt_ovrdflg
      link override Signal_Override/_ovrdval: Value=KOUTP_Country1_cnt_ovrdval
  VSYS_Country2_cnt_Inproc : FVT_lib/outp/OverrideAndLimit  SystemSampleTime=-1  VariantActivationTime=update diagram  Latency=0  AutoFrameSizeCalculation=off
      link override Signal_Limit/_maxval: Value=KOUTP_Country2_cnt_maxval
      link override Signal_Limit/_minval: Value=KOUTP_Country2_cnt_minval
      link override Signal_Override/_ovrdflg: Value=KOUTP_Country2_cnt_ovrdflg
      link override Signal_Override/_ovrdval: Value=KOUTP_Country2_cnt_ovrdval
  VSYS_CurrentNmState_enum_Inproc : FVT_lib/outp/OverrideAndLimit  SystemSampleTime=-1  VariantActivationTime=update diagram  Latency=0  AutoFrameSizeCalculation=off
      link override Signal_Limit/_maxval: Value=KOUTP_CurrentNmState_enum_maxval
      link override Signal_Limit/_minval: Value=KOUTP_CurrentNmState_enum_minval
      link override Signal_Override/_ovrdflg: Value=KOUTP_CurrentNmState_enum_ovrdflg
      link override Signal_Override/_ovrdval: Value=KOUTP_CurrentNmState_enum_ovrdval
  VSYS_Dash1_cnt_Inproc : FVT_lib/outp/OverrideAndLimit  SystemSampleTime=-1  VariantActivationTime=update diagram  Latency=0  AutoFrameSizeCalculation=off
      link override Signal_Limit/_maxval: Value=KOUTP_Dash1_cnt_maxval
      link override Signal_Limit/_minval: Value=KOUTP_Dash1_cnt_minval
      link override Signal_Override/_ovrdflg: Value=KOUTP_Dash1_cnt_ovrdflg
      link override Signal_Override/_ovrdval: Value=KOUTP_Dash1_cnt_ovrdval
  VSYS_Dash2_cnt_Inproc : FVT_lib/outp/OverrideAndLimit  SystemSampleTime=-1  VariantActivationTime=update diagram  Latency=0  AutoFrameSizeCalculation=off
      link override Signal_Limit/_maxval: Value=KOUTP_Dash2_cnt_maxval
      link override Signal_Limit/_minval: Value=KOUTP_Dash2_cnt_minval
      link override Signal_Override/_ovrdflg: Value=KOUTP_Dash2_cnt_ovrdflg
      link override Signal_Override/_ovrdval: Value=KOUTP_Dash2_cnt_ovrdval
  VSYS_ECU1_cnt_Inproc : FVT_lib/outp/OverrideAndLimit  SystemSampleTime=-1  VariantActivationTime=update diagram  Latency=0  AutoFrameSizeCalculation=off
      link override Signal_Limit/_maxval: Value=KOUTP_ECU1_cnt_maxval
      link override Signal_Limit/_minval: Value=KOUTP_ECU1_cnt_minval
      link override Signal_Override/_ovrdflg: Value=KOUTP_ECU1_cnt_ovrdflg
      link override Signal_Override/_ovrdval: Value=KOUTP_ECU1_cnt_ovrdval
  VSYS_ECU2_cnt_Inproc : FVT_lib/outp/OverrideAndLimit  SystemSampleTime=-1  VariantActivationTime=update diagram  Latency=0  AutoFrameSizeCalculation=off
      link override Signal_Limit/_maxval: Value=KOUTP_ECU2_cnt_maxval
      link override Signal_Limit/_minval: Value=KOUTP_ECU2_cnt_minval
      link override Signal_Override/_ovrdflg: Value=KOUTP_ECU2_cnt_ovrdflg
      link override Signal_Override/_ovrdval: Value=KOUTP_ECU2_cnt_ovrdval
  VSYS_FdcSlpReqRisingEdge_flg_Inproc : FVT_lib/outp/OverrideAndLimit  SystemSampleTime=-1  VariantActivationTime=update diagram  Latency=0  AutoFrameSizeCalculation=off
      link override Signal_Limit/_maxval: Value=KOUTP_FdcSlpReqRisingEdge_flg_maxval
      link override Signal_Limit/_minval: Value=KOUTP_FdcSlpReqRisingEdge_flg_minval
      link override Signal_Override/_ovrdflg: Value=KOUTP_FdcSlpReqRisingEdge_flg_ovrdflg
      link override Signal_Override/_ovrdval: Value=KOUTP_FdcSlpReqRisingEdge_flg_ovrdval
  VSYS_FdcSlpTime_sec_Inproc : FVT_lib/outp/OverrideAndLimit  SystemSampleTime=-1  VariantActivationTime=update diagram  Latency=0  AutoFrameSizeCalculation=off
      link override Signal_Limit/_maxval: Value=KOUTP_FdcSlpTime_sec_maxval
      link override Signal_Limit/_minval: Value=KOUTP_FdcSlpTime_sec_minval
      link override Signal_Override/_ovrdflg: Value=KOUTP_FdcSlpTime_sec_ovrdflg
      link override Signal_Override/_ovrdval: Value=KOUTP_FdcSlpTime_sec_ovrdval
  VSYS_HWVer1_cnt_Inproc : FVT_lib/outp/OverrideAndLimit  SystemSampleTime=-1  VariantActivationTime=update diagram  Latency=0  AutoFrameSizeCalculation=off
      link override Signal_Limit/_maxval: Value=KOUTP_HWVer1_cnt_maxval
      link override Signal_Limit/_minval: Value=KOUTP_HWVer1_cnt_minval
      link override Signal_Override/_ovrdflg: Value=KOUTP_HWVer1_cnt_ovrdflg
      link override Signal_Override/_ovrdval: Value=KOUTP_HWVer1_cnt_ovrdval
  VSYS_HWVer2_cnt_Inproc : FVT_lib/outp/OverrideAndLimit  SystemSampleTime=-1  VariantActivationTime=update diagram  Latency=0  AutoFrameSizeCalculation=off
      link override Signal_Limit/_maxval: Value=KOUTP_HWVer2_cnt_maxval
      link override Signal_Limit/_minval: Value=KOUTP_HWVer2_cnt_minval
      link override Signal_Override/_ovrdflg: Value=KOUTP_HWVer2_cnt_ovrdflg
      link override Signal_Override/_ovrdval: Value=KOUTP_HWVer2_cnt_ovrdval
  VSYS_HWVer3_cnt_Inproc : FVT_lib/outp/OverrideAndLimit  SystemSampleTime=-1  VariantActivationTime=update diagram  Latency=0  AutoFrameSizeCalculation=off
      link override Signal_Limit/_maxval: Value=KOUTP_HWVer3_cnt_maxval
      link override Signal_Limit/_minval: Value=KOUTP_HWVer3_cnt_minval
      link override Signal_Override/_ovrdflg: Value=KOUTP_HWVer3_cnt_ovrdflg
      link override Signal_Override/_ovrdval: Value=KOUTP_HWVer3_cnt_ovrdval
  VSYS_Major1_cnt_Inproc : FVT_lib/outp/OverrideAndLimit  SystemSampleTime=-1  VariantActivationTime=update diagram  Latency=0  AutoFrameSizeCalculation=off
      link override Signal_Limit/_maxval: Value=KOUTP_Major1_cnt_maxval
      link override Signal_Limit/_minval: Value=KOUTP_Major1_cnt_minval
      link override Signal_Override/_ovrdflg: Value=KOUTP_Major1_cnt_ovrdflg
      link override Signal_Override/_ovrdval: Value=KOUTP_Major1_cnt_ovrdval
  VSYS_Major2_cnt_Inproc : FVT_lib/outp/OverrideAndLimit  SystemSampleTime=-1  VariantActivationTime=update diagram  Latency=0  AutoFrameSizeCalculation=off
      link override Signal_Limit/_maxval: Value=KOUTP_Major2_cnt_maxval
      link override Signal_Limit/_minval: Value=KOUTP_Major2_cnt_minval
      link override Signal_Override/_ovrdflg: Value=KOUTP_Major2_cnt_ovrdflg
      link override Signal_Override/_ovrdval: Value=KOUTP_Major2_cnt_ovrdval
  VSYS_Minor1_cnt_Inproc : FVT_lib/outp/OverrideAndLimit  SystemSampleTime=-1  VariantActivationTime=update diagram  Latency=0  AutoFrameSizeCalculation=off
      link override Signal_Limit/_maxval: Value=KOUTP_Minor1_cnt_maxval
      link override Signal_Limit/_minval: Value=KOUTP_Minor1_cnt_minval
      link override Signal_Override/_ovrdflg: Value=KOUTP_Minor1_cnt_ovrdflg
      link override Signal_Override/_ovrdval: Value=KOUTP_Minor1_cnt_ovrdval
  VSYS_Minor2_cnt_Inproc : FVT_lib/outp/OverrideAndLimit  SystemSampleTime=-1  VariantActivationTime=update diagram  Latency=0  AutoFrameSizeCalculation=off
      link override Signal_Limit/_maxval: Value=KOUTP_Minor2_cnt_maxval
      link override Signal_Limit/_minval: Value=KOUTP_Minor2_cnt_minval
      link override Signal_Override/_ovrdflg: Value=KOUTP_Minor2_cnt_ovrdflg
      link override Signal_Override/_ovrdval: Value=KOUTP_Minor2_cnt_ovrdval
  VSYS_NvWriteReqRisingEdge_flg_Inproc : FVT_lib/outp/OverrideAndLimit  SystemSampleTime=-1  VariantActivationTime=update diagram  Latency=0  AutoFrameSizeCalculation=off
      link override Signal_Limit/_maxval: Value=KOUTP_NvWriteReqRisingEdge_flg_maxval
      link override Signal_Limit/_minval: Value=KOUTP_NvWriteReqRisingEdge_flg_minval
      link override Signal_Override/_ovrdflg: Value=KOUTP_NvWriteReqRisingEdge_flg_ovrdflg
      link override Signal_Override/_ovrdval: Value=KOUTP_NvWriteReqRisingEdge_flg_ovrdval
  VSYS_Patch1_cnt_Inproc : FVT_lib/outp/OverrideAndLimit  SystemSampleTime=-1  VariantActivationTime=update diagram  Latency=0  AutoFrameSizeCalculation=off
      link override Signal_Limit/_maxval: Value=KOUTP_Patch1_cnt_maxval
      link override Signal_Limit/_minval: Value=KOUTP_Patch1_cnt_minval
      link override Signal_Override/_ovrdflg: Value=KOUTP_Patch1_cnt_ovrdflg
      link override Signal_Override/_ovrdval: Value=KOUTP_Patch1_cnt_ovrdval
  VSYS_Patch2_cnt_Inproc : FVT_lib/outp/OverrideAndLimit  SystemSampleTime=-1  VariantActivationTime=update diagram  Latency=0  AutoFrameSizeCalculation=off
      link override Signal_Limit/_maxval: Value=KOUTP_Patch2_cnt_maxval
      link override Signal_Limit/_minval: Value=KOUTP_Patch2_cnt_minval
      link override Signal_Override/_ovrdflg: Value=KOUTP_Patch2_cnt_ovrdflg
      link override Signal_Override/_ovrdval: Value=KOUTP_Patch2_cnt_ovrdval
  VSYS_PmicBootReason_enum_Inproc : FVT_lib/outp/OverrideAndLimit  SystemSampleTime=-1  VariantActivationTime=update diagram  Latency=0  AutoFrameSizeCalculation=off
      link override Signal_Limit/_maxval: Value=KOUTP_PmicBootReason_enum_maxval
      link override Signal_Limit/_minval: Value=KOUTP_PmicBootReason_enum_minval
      link override Signal_Override/_ovrdflg: Value=KOUTP_PmicBootReason_enum_ovrdflg
      link override Signal_Override/_ovrdval: Value=KOUTP_PmicBootReason_enum_ovrdval
  VSYS_SHA1_cnt_Inproc : FVT_lib/outp/OverrideAndLimit  SystemSampleTime=-1  VariantActivationTime=update diagram  Latency=0  AutoFrameSizeCalculation=off
      link override Signal_Limit/_maxval: Value=KOUTP_SHA1_cnt_maxval
      link override Signal_Limit/_minval: Value=KOUTP_SHA1_cnt_minval
      link override Signal_Override/_ovrdflg: Value=KOUTP_SHA1_cnt_ovrdflg
      link override Signal_Override/_ovrdval: Value=KOUTP_SHA1_cnt_ovrdval
  VSYS_SHA2_cnt_Inproc : FVT_lib/outp/OverrideAndLimit  SystemSampleTime=-1  VariantActivationTime=update diagram  Latency=0  AutoFrameSizeCalculation=off
      link override Signal_Limit/_maxval: Value=KOUTP_SHA2_cnt_maxval
      link override Signal_Limit/_minval: Value=KOUTP_SHA2_cnt_minval
      link override Signal_Override/_ovrdflg: Value=KOUTP_SHA2_cnt_ovrdflg
      link override Signal_Override/_ovrdval: Value=KOUTP_SHA2_cnt_ovrdval
  VSYS_SHA3_cnt_Inproc : FVT_lib/outp/OverrideAndLimit  SystemSampleTime=-1  VariantActivationTime=update diagram  Latency=0  AutoFrameSizeCalculation=off
      link override Signal_Limit/_maxval: Value=KOUTP_SHA3_cnt_maxval
      link override Signal_Limit/_minval: Value=KOUTP_SHA3_cnt_minval
      link override Signal_Override/_ovrdflg: Value=KOUTP_SHA3_cnt_ovrdflg
      link override Signal_Override/_ovrdval: Value=KOUTP_SHA3_cnt_ovrdval
  VSYS_SHA4_cnt_Inproc : FVT_lib/outp/OverrideAndLimit  SystemSampleTime=-1  VariantActivationTime=update diagram  Latency=0  AutoFrameSizeCalculation=off
      link override Signal_Limit/_maxval: Value=KOUTP_SHA4_cnt_maxval
      link override Signal_Limit/_minval: Value=KOUTP_SHA4_cnt_minval
      link override Signal_Override/_ovrdflg: Value=KOUTP_SHA4_cnt_ovrdflg
      link override Signal_Override/_ovrdval: Value=KOUTP_SHA4_cnt_ovrdval
  VSYS_SHA5_cnt_Inproc : FVT_lib/outp/OverrideAndLimit  SystemSampleTime=-1  VariantActivationTime=update diagram  Latency=0  AutoFrameSizeCalculation=off
      link override Signal_Limit/_maxval: Value=KOUTP_SHA5_cnt_maxval
      link override Signal_Limit/_minval: Value=KOUTP_SHA5_cnt_minval
      link override Signal_Override/_ovrdflg: Value=KOUTP_SHA5_cnt_ovrdflg
      link override Signal_Override/_ovrdval: Value=KOUTP_SHA5_cnt_ovrdval
  VSYS_SHA6_cnt_Inproc : FVT_lib/outp/OverrideAndLimit  SystemSampleTime=-1  VariantActivationTime=update diagram  Latency=0  AutoFrameSizeCalculation=off
      link override Signal_Limit/_maxval: Value=KOUTP_SHA6_cnt_maxval
      link override Signal_Limit/_minval: Value=KOUTP_SHA6_cnt_minval
      link override Signal_Override/_ovrdflg: Value=KOUTP_SHA6_cnt_ovrdflg
      link override Signal_Override/_ovrdval: Value=KOUTP_SHA6_cnt_ovrdval
  VSYS_SHA7_cnt_Inproc : FVT_lib/outp/OverrideAndLimit  SystemSampleTime=-1  VariantActivationTime=update diagram  Latency=0  AutoFrameSizeCalculation=off
      link override Signal_Limit/_maxval: Value=KOUTP_SHA7_cnt_maxval
      link override Signal_Limit/_minval: Value=KOUTP_SHA7_cnt_minval
      link override Signal_Override/_ovrdflg: Value=KOUTP_SHA7_cnt_ovrdflg
      link override Signal_Override/_ovrdval: Value=KOUTP_SHA7_cnt_ovrdval
  VSYS_SHA8_cnt_Inproc : FVT_lib/outp/OverrideAndLimit  SystemSampleTime=-1  VariantActivationTime=update diagram  Latency=0  AutoFrameSizeCalculation=off
      link override Signal_Limit/_maxval: Value=KOUTP_SHA8_cnt_maxval
      link override Signal_Limit/_minval: Value=KOUTP_SHA8_cnt_minval
      link override Signal_Override/_ovrdflg: Value=KOUTP_SHA8_cnt_ovrdflg
      link override Signal_Override/_ovrdval: Value=KOUTP_SHA8_cnt_ovrdval
  VSYS_Variation_cnt_Inproc : FVT_lib/outp/OverrideAndLimit  SystemSampleTime=-1  VariantActivationTime=update diagram  Latency=0  AutoFrameSizeCalculation=off
      link override Signal_Limit/_maxval: Value=KOUTP_Variation_cnt_maxval
      link override Signal_Limit/_minval: Value=KOUTP_Variation_cnt_minval
      link override Signal_Override/_ovrdflg: Value=KOUTP_Variation_cnt_ovrdflg
      link override Signal_Override/_ovrdval: Value=KOUTP_Variation_cnt_ovrdval
  VSYS_WisrBootReason_raw32_Inproc : FVT_lib/outp/OverrideAndLimit  SystemSampleTime=-1  VariantActivationTime=update diagram  Latency=0  AutoFrameSizeCalculation=off
      link override Signal_Limit/_maxval: Value=KOUTP_WisrBootReason_raw32_maxval
      link override Signal_Limit/_minval: Value=KOUTP_WisrBootReason_raw32_minval
      link override Signal_Override/_ovrdflg: Value=KOUTP_WisrBootReason_raw32_ovrdflg
      link override Signal_Override/_ovrdval: Value=KOUTP_WisrBootReason_raw32_ovrdval
  VTHC_ACForceOFF_flg_Inproc : FVT_lib/outp/OverrideAndLimit  SystemSampleTime=-1  VariantActivationTime=update diagram  Latency=0  AutoFrameSizeCalculation=off
      link override Signal_Limit/_maxval: Value=KOUTP_ACForceOFF_flg_maxval
      link override Signal_Limit/_minval: Value=KOUTP_ACForceOFF_flg_minval
      link override Signal_Override/_ovrdflg: Value=KOUTP_ACForceOFF_flg_ovrdflg
      link override Signal_Override/_ovrdval: Value=KOUTP_ACForceOFF_flg_ovrdval
  VTHC_ACModeMem_enum_Inproc : FVT_lib/outp/OverrideAndLimit  SystemSampleTime=-1  VariantActivationTime=update diagram  Latency=0  AutoFrameSizeCalculation=off
      link override Signal_Limit/_maxval: Value=KOUTP_ACModeMem_enum_maxval
      link override Signal_Limit/_minval: Value=KOUTP_ACModeMem_enum_minval
      link override Signal_Override/_ovrdflg: Value=KOUTP_ACModeMem_enum_ovrdflg
      link override Signal_Override/_ovrdval: Value=KOUTP_ACModeMem_enum_ovrdval
  VTHC_ACSubMode_enum_Inproc : FVT_lib/outp/OverrideAndLimit  SystemSampleTime=-1  VariantActivationTime=update diagram  Latency=0  AutoFrameSizeCalculation=off
      link override Signal_Limit/_maxval: Value=KOUTP_ACSubMode_enum_maxval
      link override Signal_Limit/_minval: Value=KOUTP_ACSubMode_enum_minval
      link override Signal_Override/_ovrdflg: Value=KOUTP_ACSubMode_enum_ovrdflg
      link override Signal_Override/_ovrdval: Value=KOUTP_ACSubMode_enum_ovrdval
  VTHC_AirIntenZone1M_enum_Inproc : FVT_lib/outp/OverrideAndLimit  SystemSampleTime=-1  VariantActivationTime=update diagram  Latency=0  AutoFrameSizeCalculation=off
      link override Signal_Limit/_maxval: Value=KOUTP_AirIntenZone1M_enum_maxval
      link override Signal_Limit/_minval: Value=KOUTP_AirIntenZone1M_enum_minval
      link override Signal_Override/_ovrdflg: Value=KOUTP_AirIntenZone1M_enum_ovrdflg
      link override Signal_Override/_ovrdval: Value=KOUTP_AirIntenZone1M_enum_ovrdval
  VTHC_BatteryMode_enum_Inproc : FVT_lib/outp/OverrideAndLimit  SystemSampleTime=-1  VariantActivationTime=update diagram  Latency=0  AutoFrameSizeCalculation=off
      link override Signal_Limit/_maxval: Value=KOUTP_BatteryMode_enum_maxval
      link override Signal_Limit/_minval: Value=KOUTP_BatteryMode_enum_minval
      link override Signal_Override/_ovrdflg: Value=KOUTP_BatteryMode_enum_ovrdflg
      link override Signal_Override/_ovrdval: Value=KOUTP_BatteryMode_enum_ovrdval
  VTHC_CCUACLampSts_flg_Inproc : FVT_lib/outp/OverrideAndLimit  SystemSampleTime=-1  VariantActivationTime=update diagram  Latency=0  AutoFrameSizeCalculation=off
      link override Signal_Limit/_maxval: Value=KOUTP_CCUACLampSts_flg_maxval
      link override Signal_Limit/_minval: Value=KOUTP_CCUACLampSts_flg_minval
      link override Signal_Override/_ovrdflg: Value=KOUTP_CCUACLampSts_flg_ovrdflg
      link override Signal_Override/_ovrdval: Value=KOUTP_CCUACLampSts_flg_ovrdval
  VTHC_CCUACMaxLampSts_flg_Inproc : FVT_lib/outp/OverrideAndLimit  SystemSampleTime=-1  VariantActivationTime=update diagram  Latency=0  AutoFrameSizeCalculation=off
      link override Signal_Limit/_maxval: Value=KOUTP_CCUACMaxLampSts_flg_maxval
      link override Signal_Limit/_minval: Value=KOUTP_CCUACMaxLampSts_flg_minval
      link override Signal_Override/_ovrdflg: Value=KOUTP_CCUACMaxLampSts_flg_ovrdflg
      link override Signal_Override/_ovrdval: Value=KOUTP_CCUACMaxLampSts_flg_ovrdval
  VTHC_CCUAutoLampSts_flg_Inproc : FVT_lib/outp/OverrideAndLimit  SystemSampleTime=-1  VariantActivationTime=update diagram  Latency=0  AutoFrameSizeCalculation=off
      link override Signal_Limit/_maxval: Value=KOUTP_CCUAutoLampSts_flg_maxval
      link override Signal_Limit/_minval: Value=KOUTP_CCUAutoLampSts_flg_minval
      link override Signal_Override/_ovrdflg: Value=KOUTP_CCUAutoLampSts_flg_ovrdflg
      link override Signal_Override/_ovrdval: Value=KOUTP_CCUAutoLampSts_flg_ovrdval
  VTHC_CCUSyncLampSts_flg_Inproc : FVT_lib/outp/OverrideAndLimit  SystemSampleTime=-1  VariantActivationTime=update diagram  Latency=0  AutoFrameSizeCalculation=off
      link override Signal_Limit/_maxval: Value=KOUTP_CCUSyncLampSts_flg_maxval
      link override Signal_Limit/_minval: Value=KOUTP_CCUSyncLampSts_flg_minval
      link override Signal_Override/_ovrdflg: Value=KOUTP_CCUSyncLampSts_flg_ovrdflg
      link override Signal_Override/_ovrdval: Value=KOUTP_CCUSyncLampSts_flg_ovrdval
  VTHC_CCUSyncSts_flg_Inproc : FVT_lib/outp/OverrideAndLimit  SystemSampleTime=-1  VariantActivationTime=update diagram  Latency=0  AutoFrameSizeCalculation=off
      link override Signal_Limit/_maxval: Value=KOUTP_CCUSyncSts_flg_maxval
      link override Signal_Limit/_minval: Value=KOUTP_CCUSyncSts_flg_minval
      link override Signal_Override/_ovrdflg: Value=KOUTP_CCUSyncSts_flg_ovrdflg
      link override Signal_Override/_ovrdval: Value=KOUTP_CCUSyncSts_flg_ovrdval
  VTHC_CabinMode_enum_Inproc : FVT_lib/outp/OverrideAndLimit  SystemSampleTime=-1  VariantActivationTime=update diagram  Latency=0  AutoFrameSizeCalculation=off
      link override Signal_Limit/_maxval: Value=KOUTP_CabinMode_enum_maxval
      link override Signal_Limit/_minval: Value=KOUTP_CabinMode_enum_minval
      link override Signal_Override/_ovrdflg: Value=KOUTP_CabinMode_enum_ovrdflg
      link override Signal_Override/_ovrdval: Value=KOUTP_CabinMode_enum_ovrdval
  VTHC_CoolgFanActDuty_pct_Inproc : FVT_lib/outp/OverrideAndLimit  SystemSampleTime=-1  VariantActivationTime=update diagram  Latency=0  AutoFrameSizeCalculation=off
      link override Signal_Limit/_maxval: Value=KOUTP_CoolgFanActDuty_pct_maxval
      link override Signal_Limit/_minval: Value=KOUTP_CoolgFanActDuty_pct_minval
      link override Signal_Override/_ovrdflg: Value=KOUTP_CoolgFanActDuty_pct_ovrdflg
      link override Signal_Override/_ovrdval: Value=KOUTP_CoolgFanActDuty_pct_ovrdval
  VTHC_EDriveMode_enum_Inproc : FVT_lib/outp/OverrideAndLimit  SystemSampleTime=-1  VariantActivationTime=update diagram  Latency=0  AutoFrameSizeCalculation=off
      link override Signal_Limit/_maxval: Value=KOUTP_EDriveMode_enum_maxval
      link override Signal_Limit/_minval: Value=KOUTP_EDriveMode_enum_minval
      link override Signal_Override/_ovrdflg: Value=KOUTP_EDriveMode_enum_ovrdflg
      link override Signal_Override/_ovrdval: Value=KOUTP_EDriveMode_enum_ovrdval
  VTHC_FDAGSCmd_enum_Inproc : FVT_lib/outp/OverrideAndLimit  SystemSampleTime=-1  VariantActivationTime=update diagram  Latency=0  AutoFrameSizeCalculation=off
      link override Signal_Limit/_maxval: Value=KOUTP_FDAGSCmd_enum_maxval
      link override Signal_Limit/_minval: Value=KOUTP_FDAGSCmd_enum_minval
      link override Signal_Override/_ovrdflg: Value=KOUTP_FDAGSCmd_enum_ovrdflg
      link override Signal_Override/_ovrdval: Value=KOUTP_FDAGSCmd_enum_ovrdval
  VTHC_FDBlowerCmd_pct_Inproc : FVT_lib/outp/OverrideAndLimit  SystemSampleTime=-1  VariantActivationTime=update diagram  Latency=0  AutoFrameSizeCalculation=off
      link override Signal_Limit/_maxval: Value=KOUTP_FDBlowerCmd_pct_maxval
      link override Signal_Limit/_minval: Value=KOUTP_FDBlowerCmd_pct_minval
      link override Signal_Override/_ovrdflg: Value=KOUTP_FDBlowerCmd_pct_ovrdflg
      link override Signal_Override/_ovrdval: Value=KOUTP_FDBlowerCmd_pct_ovrdval
  VTHC_FDCTHCMAPTCWarningSta_flg_Inproc : FVT_lib/outp/OverrideAndLimit  SystemSampleTime=-1  VariantActivationTime=update diagram  Latency=0  AutoFrameSizeCalculation=off
      link override Signal_Limit/_maxval: Value=KOUTP_FDCTHCMAPTCWarningSta_flg_maxval
      link override Signal_Limit/_minval: Value=KOUTP_FDCTHCMAPTCWarningSta_flg_minval
      link override Signal_Override/_ovrdflg: Value=KOUTP_FDCTHCMAPTCWarningSta_flg_ovrdflg
      link override Signal_Override/_ovrdval: Value=KOUTP_FDCTHCMAPTCWarningSta_flg_ovrdval
  VTHC_FDCompCmd_rpm_Inproc : FVT_lib/outp/OverrideAndLimit  SystemSampleTime=-1  VariantActivationTime=update diagram  Latency=0  AutoFrameSizeCalculation=off
      link override Signal_Limit/_maxval: Value=KOUTP_FDCompCmd_rpm_maxval
      link override Signal_Limit/_minval: Value=KOUTP_FDCompCmd_rpm_minval
      link override Signal_Override/_ovrdflg: Value=KOUTP_FDCompCmd_rpm_ovrdflg
      link override Signal_Override/_ovrdval: Value=KOUTP_FDCompCmd_rpm_ovrdval
  VTHC_FDEWP1Cmd_enum_Inproc : FVT_lib/outp/OverrideAndLimit  SystemSampleTime=-1  VariantActivationTime=update diagram  Latency=0  AutoFrameSizeCalculation=off
      link override Signal_Limit/_maxval: Value=KOUTP_FDEWP1Cmd_enum_maxval
      link override Signal_Limit/_minval: Value=KOUTP_FDEWP1Cmd_enum_minval
      link override Signal_Override/_ovrdflg: Value=KOUTP_FDEWP1Cmd_enum_ovrdflg
      link override Signal_Override/_ovrdval: Value=KOUTP_FDEWP1Cmd_enum_ovrdval
  VTHC_FDEWP2Cmd_enum_Inproc : FVT_lib/outp/OverrideAndLimit  SystemSampleTime=-1  VariantActivationTime=update diagram  Latency=0  AutoFrameSizeCalculation=off
      link override Signal_Limit/_maxval: Value=KOUTP_FDEWP2Cmd_enum_maxval
      link override Signal_Limit/_minval: Value=KOUTP_FDEWP2Cmd_enum_minval
      link override Signal_Override/_ovrdflg: Value=KOUTP_FDEWP2Cmd_enum_ovrdflg
      link override Signal_Override/_ovrdval: Value=KOUTP_FDEWP2Cmd_enum_ovrdval
  VTHC_FDEWP3Cmd_enum_Inproc : FVT_lib/outp/OverrideAndLimit  SystemSampleTime=-1  VariantActivationTime=update diagram  Latency=0  AutoFrameSizeCalculation=off
      link override Signal_Limit/_maxval: Value=KOUTP_FDEWP3Cmd_enum_maxval
      link override Signal_Limit/_minval: Value=KOUTP_FDEWP3Cmd_enum_minval
      link override Signal_Override/_ovrdflg: Value=KOUTP_FDEWP3Cmd_enum_ovrdflg
      link override Signal_Override/_ovrdval: Value=KOUTP_FDEWP3Cmd_enum_ovrdval
  VTHC_FDEXV1Cmd_step_Inproc : FVT_lib/outp/OverrideAndLimit  SystemSampleTime=-1  VariantActivationTime=update diagram  Latency=0  AutoFrameSizeCalculation=off
      link override Signal_Limit/_maxval: Value=KOUTP_FDEXV1Cmd_step_maxval
      link override Signal_Limit/_minval: Value=KOUTP_FDEXV1Cmd_step_minval
      link override Signal_Override/_ovrdflg: Value=KOUTP_FDEXV1Cmd_step_ovrdflg
      link override Signal_Override/_ovrdval: Value=KOUTP_FDEXV1Cmd_step_ovrdval
  VTHC_FDEXV2Cmd_step_Inproc : FVT_lib/outp/OverrideAndLimit  SystemSampleTime=-1  VariantActivationTime=update diagram  Latency=0  AutoFrameSizeCalculation=off
      link override Signal_Limit/_maxval: Value=KOUTP_FDEXV2Cmd_step_maxval
      link override Signal_Limit/_minval: Value=KOUTP_FDEXV2Cmd_step_minval
      link override Signal_Override/_ovrdflg: Value=KOUTP_FDEXV2Cmd_step_ovrdflg
      link override Signal_Override/_ovrdval: Value=KOUTP_FDEXV2Cmd_step_ovrdval
  VTHC_FDFWVCmd_flg_Inproc : FVT_lib/outp/OverrideAndLimit  SystemSampleTime=-1  VariantActivationTime=update diagram  Latency=0  AutoFrameSizeCalculation=off
      link override Signal_Limit/_maxval: Value=KOUTP_FDFWVCmd_flg_maxval
      link override Signal_Limit/_minval: Value=KOUTP_FDFWVCmd_flg_minval
      link override Signal_Override/_ovrdflg: Value=KOUTP_FDFWVCmd_flg_ovrdflg
      link override Signal_Override/_ovrdval: Value=KOUTP_FDFWVCmd_flg_ovrdval
  VTHC_FDFrLeAPTCHeatPwrCmd_W_Inproc : FVT_lib/outp/OverrideAndLimit  SystemSampleTime=-1  VariantActivationTime=update diagram  Latency=0  AutoFrameSizeCalculation=off
      link override Signal_Limit/_maxval: Value=KOUTP_FDFrLeAPTCHeatPwrCmd_W_maxval
      link override Signal_Limit/_minval: Value=KOUTP_FDFrLeAPTCHeatPwrCmd_W_minval
      link override Signal_Override/_ovrdflg: Value=KOUTP_FDFrLeAPTCHeatPwrCmd_W_ovrdflg
      link override Signal_Override/_ovrdval: Value=KOUTP_FDFrLeAPTCHeatPwrCmd_W_ovrdval
  VTHC_FDFrRiAPTCHeatPwrCmd_W_Inproc : FVT_lib/outp/OverrideAndLimit  SystemSampleTime=-1  VariantActivationTime=update diagram  Latency=0  AutoFrameSizeCalculation=off
      link override Signal_Limit/_maxval: Value=KOUTP_FDFrRiAPTCHeatPwrCmd_W_maxval
      link override Signal_Limit/_minval: Value=KOUTP_FDFrRiAPTCHeatPwrCmd_W_minval
      link override Signal_Override/_ovrdflg: Value=KOUTP_FDFrRiAPTCHeatPwrCmd_W_ovrdflg
      link override Signal_Override/_ovrdval: Value=KOUTP_FDFrRiAPTCHeatPwrCmd_W_ovrdval
  VTHC_FDFrWPTCHeatPwrCmd_W_Inproc : FVT_lib/outp/OverrideAndLimit  SystemSampleTime=-1  VariantActivationTime=update diagram  Latency=0  AutoFrameSizeCalculation=off
      link override Signal_Limit/_maxval: Value=KOUTP_FDFrWPTCHeatPwrCmd_W_maxval
      link override Signal_Limit/_minval: Value=KOUTP_FDFrWPTCHeatPwrCmd_W_minval
      link override Signal_Override/_ovrdflg: Value=KOUTP_FDFrWPTCHeatPwrCmd_W_ovrdflg
      link override Signal_Override/_ovrdval: Value=KOUTP_FDFrWPTCHeatPwrCmd_W_ovrdval
  VTHC_FDRecyAutoCmd_enum_Inproc : FVT_lib/outp/OverrideAndLimit  SystemSampleTime=-1  VariantActivationTime=update diagram  Latency=0  AutoFrameSizeCalculation=off
      link override Signal_Limit/_maxval: Value=KOUTP_FDRecyAutoCmd_enum_maxval
      link override Signal_Limit/_minval: Value=KOUTP_FDRecyAutoCmd_enum_minval
      link override Signal_Override/_ovrdflg: Value=KOUTP_FDRecyAutoCmd_enum_ovrdflg
      link override Signal_Override/_ovrdval: Value=KOUTP_FDRecyAutoCmd_enum_ovrdval
  VTHC_FDRrAPTCHeatPwrCmd_W_Inproc : FVT_lib/outp/OverrideAndLimit  SystemSampleTime=-1  VariantActivationTime=update diagram  Latency=0  AutoFrameSizeCalculation=off
      link override Signal_Limit/_maxval: Value=KOUTP_FDRrAPTCHeatPwrCmd_W_maxval
      link override Signal_Limit/_minval: Value=KOUTP_FDRrAPTCHeatPwrCmd_W_minval
      link override Signal_Override/_ovrdflg: Value=KOUTP_FDRrAPTCHeatPwrCmd_W_ovrdflg
      link override Signal_Override/_ovrdval: Value=KOUTP_FDRrAPTCHeatPwrCmd_W_ovrdval
  VTHC_FDSOTXVCmd_flg_Inproc : FVT_lib/outp/OverrideAndLimit  SystemSampleTime=-1  VariantActivationTime=update diagram  Latency=0  AutoFrameSizeCalculation=off
      link override Signal_Limit/_maxval: Value=KOUTP_FDSOTXVCmd_flg_maxval
      link override Signal_Limit/_minval: Value=KOUTP_FDSOTXVCmd_flg_minval
      link override Signal_Override/_ovrdflg: Value=KOUTP_FDSOTXVCmd_flg_ovrdflg
      link override Signal_Override/_ovrdval: Value=KOUTP_FDSOTXVCmd_flg_ovrdval
  VTHC_FDSOV1Cmd_flg_Inproc : FVT_lib/outp/OverrideAndLimit  SystemSampleTime=-1  VariantActivationTime=update diagram  Latency=0  AutoFrameSizeCalculation=off
      link override Signal_Limit/_maxval: Value=KOUTP_FDSOV1Cmd_flg_maxval
      link override Signal_Limit/_minval: Value=KOUTP_FDSOV1Cmd_flg_minval
      link override Signal_Override/_ovrdflg: Value=KOUTP_FDSOV1Cmd_flg_ovrdflg
      link override Signal_Override/_ovrdval: Value=KOUTP_FDSOV1Cmd_flg_ovrdval
  VTHC_FDSOV2Cmd_flg_Inproc : FVT_lib/outp/OverrideAndLimit  SystemSampleTime=-1  VariantActivationTime=update diagram  Latency=0  AutoFrameSizeCalculation=off
      link override Signal_Limit/_maxval: Value=KOUTP_FDSOV2Cmd_flg_maxval
      link override Signal_Limit/_minval: Value=KOUTP_FDSOV2Cmd_flg_minval
      link override Signal_Override/_ovrdflg: Value=KOUTP_FDSOV2Cmd_flg_ovrdflg
      link override Signal_Override/_ovrdval: Value=KOUTP_FDSOV2Cmd_flg_ovrdval
  VTHC_FDSOV3Cmd_flg_Inproc : FVT_lib/outp/OverrideAndLimit  SystemSampleTime=-1  VariantActivationTime=update diagram  Latency=0  AutoFrameSizeCalculation=off
      link override Signal_Limit/_maxval: Value=KOUTP_FDSOV3Cmd_flg_maxval
      link override Signal_Limit/_minval: Value=KOUTP_FDSOV3Cmd_flg_minval
      link override Signal_Override/_ovrdflg: Value=KOUTP_FDSOV3Cmd_flg_ovrdflg
      link override Signal_Override/_ovrdval: Value=KOUTP_FDSOV3Cmd_flg_ovrdval
  VTHC_FDTWVCmd_pct_Inproc : FVT_lib/outp/OverrideAndLimit  SystemSampleTime=-1  VariantActivationTime=update diagram  Latency=0  AutoFrameSizeCalculation=off
      link override Signal_Limit/_maxval: Value=KOUTP_FDTWVCmd_pct_maxval
      link override Signal_Limit/_minval: Value=KOUTP_FDTWVCmd_pct_minval
      link override Signal_Override/_ovrdflg: Value=KOUTP_FDTWVCmd_pct_ovrdflg
      link override Signal_Override/_ovrdval: Value=KOUTP_FDTWVCmd_pct_ovrdval
  VTHC_FaceM_flg_Inproc : FVT_lib/outp/OverrideAndLimit  SystemSampleTime=-1  VariantActivationTime=update diagram  Latency=0  AutoFrameSizeCalculation=off
      link override Signal_Limit/_maxval: Value=KOUTP_FaceM_flg_maxval
      link override Signal_Limit/_minval: Value=KOUTP_FaceM_flg_minval
      link override Signal_Override/_ovrdflg: Value=KOUTP_FaceM_flg_ovrdflg
      link override Signal_Override/_ovrdval: Value=KOUTP_FaceM_flg_ovrdval
  VTHC_Face_flg_Inproc : FVT_lib/outp/OverrideAndLimit  SystemSampleTime=-1  VariantActivationTime=update diagram  Latency=0  AutoFrameSizeCalculation=off
      link override Signal_Limit/_maxval: Value=KOUTP_Face_flg_maxval
      link override Signal_Limit/_minval: Value=KOUTP_Face_flg_minval
      link override Signal_Override/_ovrdflg: Value=KOUTP_Face_flg_ovrdflg
      link override Signal_Override/_ovrdval: Value=KOUTP_Face_flg_ovrdval
  VTHC_FootM_flg_Inproc : FVT_lib/outp/OverrideAndLimit  SystemSampleTime=-1  VariantActivationTime=update diagram  Latency=0  AutoFrameSizeCalculation=off
      link override Signal_Limit/_maxval: Value=KOUTP_FootM_flg_maxval
      link override Signal_Limit/_minval: Value=KOUTP_FootM_flg_minval
      link override Signal_Override/_ovrdflg: Value=KOUTP_FootM_flg_ovrdflg
      link override Signal_Override/_ovrdval: Value=KOUTP_FootM_flg_ovrdval
  VTHC_Foot_flg_Inproc : FVT_lib/outp/OverrideAndLimit  SystemSampleTime=-1  VariantActivationTime=update diagram  Latency=0  AutoFrameSizeCalculation=off
      link override Signal_Limit/_maxval: Value=KOUTP_Foot_flg_maxval
      link override Signal_Limit/_minval: Value=KOUTP_Foot_flg_minval
      link override Signal_Override/_ovrdflg: Value=KOUTP_Foot_flg_ovrdflg
      link override Signal_Override/_ovrdval: Value=KOUTP_Foot_flg_ovrdval
  VTHC_Frost_flg_Inproc : FVT_lib/outp/OverrideAndLimit  SystemSampleTime=-1  VariantActivationTime=update diagram  Latency=0  AutoFrameSizeCalculation=off
      link override Signal_Limit/_maxval: Value=KOUTP_Frost_flg_maxval
      link override Signal_Limit/_minval: Value=KOUTP_Frost_flg_minval
      link override Signal_Override/_ovrdflg: Value=KOUTP_Frost_flg_ovrdflg
      link override Signal_Override/_ovrdval: Value=KOUTP_Frost_flg_ovrdval
  VTHC_RecAutoFlg_flg_Inproc : FVT_lib/outp/OverrideAndLimit  SystemSampleTime=-1  VariantActivationTime=update diagram  Latency=0  AutoFrameSizeCalculation=off
      link override Signal_Limit/_maxval: Value=KOUTP_RecAutoFlg_flg_maxval
      link override Signal_Limit/_minval: Value=KOUTP_RecAutoFlg_flg_minval
      link override Signal_Override/_ovrdflg: Value=KOUTP_RecAutoFlg_flg_ovrdflg
      link override Signal_Override/_ovrdval: Value=KOUTP_RecAutoFlg_flg_ovrdval
  VTHC_fdefog_flg_Inproc : FVT_lib/outp/OverrideAndLimit  SystemSampleTime=-1  VariantActivationTime=update diagram  Latency=0  AutoFrameSizeCalculation=off
      link override Signal_Limit/_maxval: Value=KOUTP_fdefog_flg_maxval
      link override Signal_Limit/_minval: Value=KOUTP_fdefog_flg_minval
      link override Signal_Override/_ovrdflg: Value=KOUTP_fdefog_flg_ovrdflg
      link override Signal_Override/_ovrdval: Value=KOUTP_fdefog_flg_ovrdval
  VTHC_sigAirIntenZon1St_enum_Inproc : FVT_lib/outp/OverrideAndLimit  SystemSampleTime=-1  VariantActivationTime=update diagram  Latency=0  AutoFrameSizeCalculation=off
      link override Signal_Limit/_maxval: Value=KOUTP_sigAirIntenZon1St_enum_maxval
      link override Signal_Limit/_minval: Value=KOUTP_sigAirIntenZon1St_enum_minval
      link override Signal_Override/_ovrdflg: Value=KOUTP_sigAirIntenZon1St_enum_ovrdflg
      link override Signal_Override/_ovrdval: Value=KOUTP_sigAirIntenZon1St_enum_ovrdval
  VTHC_sigAmbAirT_C_Inproc : FVT_lib/outp/OverrideAndLimit  SystemSampleTime=-1  VariantActivationTime=update diagram  Latency=0  AutoFrameSizeCalculation=off
      link override Signal_Limit/_maxval: Value=KOUTP_sigAmbAirT_C_maxval
      link override Signal_Limit/_minval: Value=KOUTP_sigAmbAirT_C_minval
      link override Signal_Override/_ovrdflg: Value=KOUTP_sigAmbAirT_C_ovrdflg
      link override Signal_Override/_ovrdval: Value=KOUTP_sigAmbAirT_C_ovrdval
  VTHC_sigCbnAirT_C_Inproc : FVT_lib/outp/OverrideAndLimit  SystemSampleTime=-1  VariantActivationTime=update diagram  Latency=0  AutoFrameSizeCalculation=off
      link override Signal_Limit/_maxval: Value=KOUTP_sigCbnAirT_C_maxval
      link override Signal_Limit/_minval: Value=KOUTP_sigCbnAirT_C_minval
      link override Signal_Override/_ovrdflg: Value=KOUTP_sigCbnAirT_C_ovrdflg
      link override Signal_Override/_ovrdval: Value=KOUTP_sigCbnAirT_C_ovrdval
  VTHC_sigCbnSolarLeft_W_Inproc : FVT_lib/outp/OverrideAndLimit  SystemSampleTime=-1  VariantActivationTime=update diagram  Latency=0  AutoFrameSizeCalculation=off
      link override Signal_Limit/_maxval: Value=KOUTP_sigCbnSolarLeft_W_maxval
      link override Signal_Limit/_minval: Value=KOUTP_sigCbnSolarLeft_W_minval
      link override Signal_Override/_ovrdflg: Value=KOUTP_sigCbnSolarLeft_W_ovrdflg
      link override Signal_Override/_ovrdval: Value=KOUTP_sigCbnSolarLeft_W_ovrdval
  VTHC_sigCbnSolarRight_W_Inproc : FVT_lib/outp/OverrideAndLimit  SystemSampleTime=-1  VariantActivationTime=update diagram  Latency=0  AutoFrameSizeCalculation=off
      link override Signal_Limit/_maxval: Value=KOUTP_sigCbnSolarRight_W_maxval
      link override Signal_Limit/_minval: Value=KOUTP_sigCbnSolarRight_W_minval
      link override Signal_Override/_ovrdflg: Value=KOUTP_sigCbnSolarRight_W_ovrdflg
      link override Signal_Override/_ovrdval: Value=KOUTP_sigCbnSolarRight_W_ovrdval
  VTHC_sigClntTHvBattIn_C_Inproc : FVT_lib/outp/OverrideAndLimit  SystemSampleTime=-1  VariantActivationTime=update diagram  Latency=0  AutoFrameSizeCalculation=off
      link override Signal_Limit/_maxval: Value=KOUTP_sigClntTHvBattIn_C_maxval
      link override Signal_Limit/_minval: Value=KOUTP_sigClntTHvBattIn_C_minval
      link override Signal_Override/_ovrdflg: Value=KOUTP_sigClntTHvBattIn_C_ovrdflg
      link override Signal_Override/_ovrdval: Value=KOUTP_sigClntTHvBattIn_C_ovrdval
  VTHC_sigClntTHvBattOut_C_Inproc : FVT_lib/outp/OverrideAndLimit  SystemSampleTime=-1  VariantActivationTime=update diagram  Latency=0  AutoFrameSizeCalculation=off
      link override Signal_Limit/_maxval: Value=KOUTP_sigClntTHvBattOut_C_maxval
      link override Signal_Limit/_minval: Value=KOUTP_sigClntTHvBattOut_C_minval
      link override Signal_Override/_ovrdflg: Value=KOUTP_sigClntTHvBattOut_C_ovrdflg
      link override Signal_Override/_ovrdval: Value=KOUTP_sigClntTHvBattOut_C_ovrdval
  VTHC_sigRecircSt_flg_Inproc : FVT_lib/outp/OverrideAndLimit  SystemSampleTime=-1  VariantActivationTime=update diagram  Latency=0  AutoFrameSizeCalculation=off
      link override Signal_Limit/_maxval: Value=KOUTP_sigRecircSt_flg_maxval
      link override Signal_Limit/_minval: Value=KOUTP_sigRecircSt_flg_minval
      link override Signal_Override/_ovrdflg: Value=KOUTP_sigRecircSt_flg_ovrdflg
      link override Signal_Override/_ovrdval: Value=KOUTP_sigRecircSt_flg_ovrdval
  VTHC_sigSetTempZon1St_C_Inproc : FVT_lib/outp/OverrideAndLimit  SystemSampleTime=-1  VariantActivationTime=update diagram  Latency=0  AutoFrameSizeCalculation=off
      link override Signal_Limit/_maxval: Value=KOUTP_sigSetTempZon1St_C_maxval
      link override Signal_Limit/_minval: Value=KOUTP_sigSetTempZon1St_C_minval
      link override Signal_Override/_ovrdflg: Value=KOUTP_sigSetTempZon1St_C_ovrdflg
      link override Signal_Override/_ovrdval: Value=KOUTP_sigSetTempZon1St_C_ovrdval
  VTHC_sigSetTempZon2StM_C_Inproc : FVT_lib/outp/OverrideAndLimit  SystemSampleTime=-1  VariantActivationTime=update diagram  Latency=0  AutoFrameSizeCalculation=off
      link override Signal_Limit/_maxval: Value=KOUTP_sigSetTempZon2StM_C_maxval
      link override Signal_Limit/_minval: Value=KOUTP_sigSetTempZon2StM_C_minval
      link override Signal_Override/_ovrdflg: Value=KOUTP_sigSetTempZon2StM_C_ovrdflg
      link override Signal_Override/_ovrdval: Value=KOUTP_sigSetTempZon2StM_C_ovrdval
  VTHC_sigSetTempZon2St_C_Inproc : FVT_lib/outp/OverrideAndLimit  SystemSampleTime=-1  VariantActivationTime=update diagram  Latency=0  AutoFrameSizeCalculation=off
      link override Signal_Limit/_maxval: Value=KOUTP_sigSetTempZon2St_C_maxval
      link override Signal_Limit/_minval: Value=KOUTP_sigSetTempZon2St_C_minval
      link override Signal_Override/_ovrdflg: Value=KOUTP_sigSetTempZon2St_C_ovrdflg
      link override Signal_Override/_ovrdval: Value=KOUTP_sigSetTempZon2St_C_ovrdval
  VTHC_sigWindDirZon1St_enum_Inproc : FVT_lib/outp/OverrideAndLimit  SystemSampleTime=-1  VariantActivationTime=update diagram  Latency=0  AutoFrameSizeCalculation=off
      link override Signal_Limit/_maxval: Value=KOUTP_sigWindDirZon1St_enum_maxval
      link override Signal_Limit/_minval: Value=KOUTP_sigWindDirZon1St_enum_minval
      link override Signal_Override/_ovrdflg: Value=KOUTP_sigWindDirZon1St_enum_ovrdflg
      link override Signal_Override/_ovrdval: Value=KOUTP_sigWindDirZon1St_enum_ovrdval
  VTPM_ALFin_flg_Inproc : FVT_lib/outp/OverrideAndLimit  SystemSampleTime=-1  VariantActivationTime=update diagram  Latency=0  AutoFrameSizeCalculation=off
      link override Signal_Limit/_maxval: Value=KOUTP_ALFin_flg_maxval
      link override Signal_Limit/_minval: Value=KOUTP_ALFin_flg_minval
      link override Signal_Override/_ovrdflg: Value=KOUTP_ALFin_flg_ovrdflg
      link override Signal_Override/_ovrdval: Value=KOUTP_ALFin_flg_ovrdval
  VTPM_AutoLTips_enum_Inproc : FVT_lib/outp/OverrideAndLimit  SystemSampleTime=-1  VariantActivationTime=update diagram  Latency=0  AutoFrameSizeCalculation=off
      link override Signal_Limit/_maxval: Value=KOUTP_AutoLTips_enum_maxval
      link override Signal_Limit/_minval: Value=KOUTP_AutoLTips_enum_minval
      link override Signal_Override/_ovrdflg: Value=KOUTP_AutoLTips_enum_ovrdflg
      link override Signal_Override/_ovrdval: Value=KOUTP_AutoLTips_enum_ovrdval
  VTPM_CWheelTips_enum_Inproc : FVT_lib/outp/OverrideAndLimit  SystemSampleTime=-1  VariantActivationTime=update diagram  Latency=0  AutoFrameSizeCalculation=off
      link override Signal_Limit/_maxval: Value=KOUTP_CWheelTips_enum_maxval
      link override Signal_Limit/_minval: Value=KOUTP_CWheelTips_enum_minval
      link override Signal_Override/_ovrdflg: Value=KOUTP_CWheelTips_enum_ovrdflg
      link override Signal_Override/_ovrdval: Value=KOUTP_CWheelTips_enum_ovrdval
  VTPM_ChkStorge_flg_Inproc : FVT_lib/outp/OverrideAndLimit  SystemSampleTime=-1  VariantActivationTime=update diagram  Latency=0  AutoFrameSizeCalculation=off
      link override Signal_Limit/_maxval: Value=KOUTP_ChkStorge_flg_maxval
      link override Signal_Limit/_minval: Value=KOUTP_ChkStorge_flg_minval
      link override Signal_Override/_ovrdflg: Value=KOUTP_ChkStorge_flg_ovrdflg
      link override Signal_Override/_ovrdval: Value=KOUTP_ChkStorge_flg_ovrdval
  VTPM_Chkfin_flg_Inproc : FVT_lib/outp/OverrideAndLimit  SystemSampleTime=-1  VariantActivationTime=update diagram  Latency=0  AutoFrameSizeCalculation=off
      link override Signal_Limit/_maxval: Value=KOUTP_Chkfin_flg_maxval
      link override Signal_Limit/_minval: Value=KOUTP_Chkfin_flg_minval
      link override Signal_Override/_ovrdflg: Value=KOUTP_Chkfin_flg_ovrdflg
      link override Signal_Override/_ovrdval: Value=KOUTP_Chkfin_flg_ovrdval
  VTPM_FAT_flg_Inproc : FVT_lib/outp/OverrideAndLimit  SystemSampleTime=-1  VariantActivationTime=update diagram  Latency=0  AutoFrameSizeCalculation=off
      link override Signal_Limit/_maxval: Value=KOUTP_FAT_flg_maxval
      link override Signal_Limit/_minval: Value=KOUTP_FAT_flg_minval
      link override Signal_Override/_ovrdflg: Value=KOUTP_FAT_flg_ovrdflg
      link override Signal_Override/_ovrdval: Value=KOUTP_FAT_flg_ovrdval
  VTPM_FlashIDvalid_enum_Inproc : FVT_lib/outp/OverrideAndLimit  SystemSampleTime=-1  VariantActivationTime=update diagram  Latency=0  AutoFrameSizeCalculation=off
      link override Signal_Limit/_maxval: Value=KOUTP_FlashIDvalid_enum_maxval
      link override Signal_Limit/_minval: Value=KOUTP_FlashIDvalid_enum_minval
      link override Signal_Override/_ovrdflg: Value=KOUTP_FlashIDvalid_enum_ovrdflg
      link override Signal_Override/_ovrdval: Value=KOUTP_FlashIDvalid_enum_ovrdval
  VTPM_FlashS1ID_raw_Inproc : FVT_lib/outp/OverrideAndLimit  SystemSampleTime=-1  VariantActivationTime=update diagram  Latency=0  AutoFrameSizeCalculation=off
      link override Signal_Limit/_maxval: Value=KOUTP_FlashS1ID_raw_maxval
      link override Signal_Limit/_minval: Value=KOUTP_FlashS1ID_raw_minval
      link override Signal_Override/_ovrdflg: Value=KOUTP_FlashS1ID_raw_ovrdflg
      link override Signal_Override/_ovrdval: Value=KOUTP_FlashS1ID_raw_ovrdval
  VTPM_FlashS2ID_raw_Inproc : FVT_lib/outp/OverrideAndLimit  SystemSampleTime=-1  VariantActivationTime=update diagram  Latency=0  AutoFrameSizeCalculation=off
      link override Signal_Limit/_maxval: Value=KOUTP_FlashS2ID_raw_maxval
      link override Signal_Limit/_minval: Value=KOUTP_FlashS2ID_raw_minval
      link override Signal_Override/_ovrdflg: Value=KOUTP_FlashS2ID_raw_ovrdflg
      link override Signal_Override/_ovrdval: Value=KOUTP_FlashS2ID_raw_ovrdval
  VTPM_FlashS3ID_raw_Inproc : FVT_lib/outp/OverrideAndLimit  SystemSampleTime=-1  VariantActivationTime=update diagram  Latency=0  AutoFrameSizeCalculation=off
      link override Signal_Limit/_maxval: Value=KOUTP_FlashS3ID_raw_maxval
      link override Signal_Limit/_minval: Value=KOUTP_FlashS3ID_raw_minval
      link override Signal_Override/_ovrdflg: Value=KOUTP_FlashS3ID_raw_ovrdflg
      link override Signal_Override/_ovrdval: Value=KOUTP_FlashS3ID_raw_ovrdval
  VTPM_FlashS4ID_raw_Inproc : FVT_lib/outp/OverrideAndLimit  SystemSampleTime=-1  VariantActivationTime=update diagram  Latency=0  AutoFrameSizeCalculation=off
      link override Signal_Limit/_maxval: Value=KOUTP_FlashS4ID_raw_maxval
      link override Signal_Limit/_minval: Value=KOUTP_FlashS4ID_raw_minval
      link override Signal_Override/_ovrdflg: Value=KOUTP_FlashS4ID_raw_ovrdflg
      link override Signal_Override/_ovrdval: Value=KOUTP_FlashS4ID_raw_ovrdval
  VTPM_Flashchkdatavalid_enum_Inproc : FVT_lib/outp/OverrideAndLimit  SystemSampleTime=-1  VariantActivationTime=update diagram  Latency=0  AutoFrameSizeCalculation=off
      link override Signal_Limit/_maxval: Value=KOUTP_Flashchkdatavalid_enum_maxval
      link override Signal_Limit/_minval: Value=KOUTP_Flashchkdatavalid_enum_minval
      link override Signal_Override/_ovrdflg: Value=KOUTP_Flashchkdatavalid_enum_ovrdflg
      link override Signal_Override/_ovrdval: Value=KOUTP_Flashchkdatavalid_enum_ovrdval
  VTPM_Flashdatavalid_enum_Inproc : FVT_lib/outp/OverrideAndLimit  SystemSampleTime=-1  VariantActivationTime=update diagram  Latency=0  AutoFrameSizeCalculation=off
      link override Signal_Limit/_maxval: Value=KOUTP_Flashdatavalid_enum_maxval
      link override Signal_Limit/_minval: Value=KOUTP_Flashdatavalid_enum_minval
      link override Signal_Override/_ovrdflg: Value=KOUTP_Flashdatavalid_enum_ovrdflg
      link override Signal_Override/_ovrdval: Value=KOUTP_Flashdatavalid_enum_ovrdval
  VTPM_ID1messageALTU_raw8_Inproc : FVT_lib/outp/OverrideAndLimit  SystemSampleTime=-1  VariantActivationTime=update diagram  Latency=0  AutoFrameSizeCalculation=off
      link override Signal_Limit/_maxval: Value=KOUTP_ID1messageALTU_raw8_maxval
      link override Signal_Limit/_minval: Value=KOUTP_ID1messageALTU_raw8_minval
      link override Signal_Override/_ovrdflg: Value=KOUTP_ID1messageALTU_raw8_ovrdflg
      link override Signal_Override/_ovrdval: Value=KOUTP_ID1messageALTU_raw8_ovrdval
  VTPM_ID2messageALTU_raw8_Inproc : FVT_lib/outp/OverrideAndLimit  SystemSampleTime=-1  VariantActivationTime=update diagram  Latency=0  AutoFrameSizeCalculation=off
      link override Signal_Limit/_maxval: Value=KOUTP_ID2messageALTU_raw8_maxval
      link override Signal_Limit/_minval: Value=KOUTP_ID2messageALTU_raw8_minval
      link override Signal_Override/_ovrdflg: Value=KOUTP_ID2messageALTU_raw8_ovrdflg
      link override Signal_Override/_ovrdval: Value=KOUTP_ID2messageALTU_raw8_ovrdval
  VTPM_ID3messageALTU_raw8_Inproc : FVT_lib/outp/OverrideAndLimit  SystemSampleTime=-1  VariantActivationTime=update diagram  Latency=0  AutoFrameSizeCalculation=off
      link override Signal_Limit/_maxval: Value=KOUTP_ID3messageALTU_raw8_maxval
      link override Signal_Limit/_minval: Value=KOUTP_ID3messageALTU_raw8_minval
      link override Signal_Override/_ovrdflg: Value=KOUTP_ID3messageALTU_raw8_ovrdflg
      link override Signal_Override/_ovrdval: Value=KOUTP_ID3messageALTU_raw8_ovrdval
  VTPM_ID4messageALTU_raw8_Inproc : FVT_lib/outp/OverrideAndLimit  SystemSampleTime=-1  VariantActivationTime=update diagram  Latency=0  AutoFrameSizeCalculation=off
      link override Signal_Limit/_maxval: Value=KOUTP_ID4messageALTU_raw8_maxval
      link override Signal_Limit/_minval: Value=KOUTP_ID4messageALTU_raw8_minval
      link override Signal_Override/_ovrdflg: Value=KOUTP_ID4messageALTU_raw8_ovrdflg
      link override Signal_Override/_ovrdval: Value=KOUTP_ID4messageALTU_raw8_ovrdval
  VTPM_IDin_raw32_Inproc : FVT_lib/outp/OverrideAndLimit  SystemSampleTime=-1  VariantActivationTime=update diagram  Latency=0  AutoFrameSizeCalculation=off
      link override Signal_Limit/_maxval: Value=KOUTP_IDin_raw32_maxval
      link override Signal_Limit/_minval: Value=KOUTP_IDin_raw32_minval
      link override Signal_Override/_ovrdflg: Value=KOUTP_IDin_raw32_ovrdflg
      link override Signal_Override/_ovrdval: Value=KOUTP_IDin_raw32_ovrdval
  VTPM_LFBatWarn_flg_Inproc : FVT_lib/outp/OverrideAndLimit  SystemSampleTime=-1  VariantActivationTime=update diagram  Latency=0  AutoFrameSizeCalculation=off
      link override Signal_Limit/_maxval: Value=KOUTP_LFBatWarn_flg_maxval
      link override Signal_Limit/_minval: Value=KOUTP_LFBatWarn_flg_minval
      link override Signal_Override/_ovrdflg: Value=KOUTP_LFBatWarn_flg_ovrdflg
      link override Signal_Override/_ovrdval: Value=KOUTP_LFBatWarn_flg_ovrdval
  VTPM_LFP20_raw8_Inproc : FVT_lib/outp/OverrideAndLimit  SystemSampleTime=-1  VariantActivationTime=update diagram  Latency=0  AutoFrameSizeCalculation=off
      link override Signal_Limit/_maxval: Value=KOUTP_LFP20_raw8_maxval
      link override Signal_Limit/_minval: Value=KOUTP_LFP20_raw8_minval
      link override Signal_Override/_ovrdflg: Value=KOUTP_LFP20_raw8_ovrdflg
      link override Signal_Override/_ovrdval: Value=KOUTP_LFP20_raw8_ovrdval
  VTPM_LFPindi_enum_Inproc : FVT_lib/outp/OverrideAndLimit  SystemSampleTime=-1  VariantActivationTime=update diagram  Latency=0  AutoFrameSizeCalculation=off
      link override Signal_Limit/_maxval: Value=KOUTP_LFPindi_enum_maxval
      link override Signal_Limit/_minval: Value=KOUTP_LFPindi_enum_minval
      link override Signal_Override/_ovrdflg: Value=KOUTP_LFPindi_enum_ovrdflg
      link override Signal_Override/_ovrdval: Value=KOUTP_LFPindi_enum_ovrdval
  VTPM_LFPressIndi_enum_Inproc : FVT_lib/outp/OverrideAndLimit  SystemSampleTime=-1  VariantActivationTime=update diagram  Latency=0  AutoFrameSizeCalculation=off
      link override Signal_Limit/_maxval: Value=KOUTP_LFPressIndi_enum_maxval
      link override Signal_Limit/_minval: Value=KOUTP_LFPressIndi_enum_minval
      link override Signal_Override/_ovrdflg: Value=KOUTP_LFPressIndi_enum_ovrdflg
      link override Signal_Override/_ovrdval: Value=KOUTP_LFPressIndi_enum_ovrdval
  VTPM_LFSensorFail_flg_Inproc : FVT_lib/outp/OverrideAndLimit  SystemSampleTime=-1  VariantActivationTime=update diagram  Latency=0  AutoFrameSizeCalculation=off
      link override Signal_Limit/_maxval: Value=KOUTP_LFSensorFail_flg_maxval
      link override Signal_Limit/_minval: Value=KOUTP_LFSensorFail_flg_minval
      link override Signal_Override/_ovrdflg: Value=KOUTP_LFSensorFail_flg_ovrdflg
      link override Signal_Override/_ovrdval: Value=KOUTP_LFSensorFail_flg_ovrdval
  VTPM_LFSensorMode_flg_Inproc : FVT_lib/outp/OverrideAndLimit  SystemSampleTime=-1  VariantActivationTime=update diagram  Latency=0  AutoFrameSizeCalculation=off
      link override Signal_Limit/_maxval: Value=KOUTP_LFSensorMode_flg_maxval
      link override Signal_Limit/_minval: Value=KOUTP_LFSensorMode_flg_minval
      link override Signal_Override/_ovrdflg: Value=KOUTP_LFSensorMode_flg_ovrdflg
      link override Signal_Override/_ovrdval: Value=KOUTP_LFSensorMode_flg_ovrdval
  VTPM_LFWheelDebug_flg_Inproc : FVT_lib/outp/OverrideAndLimit  SystemSampleTime=-1  VariantActivationTime=update diagram  Latency=0  AutoFrameSizeCalculation=off
      link override Signal_Limit/_maxval: Value=KOUTP_LFWheelDebug_flg_maxval
      link override Signal_Limit/_minval: Value=KOUTP_LFWheelDebug_flg_minval
      link override Signal_Override/_ovrdflg: Value=KOUTP_LFWheelDebug_flg_ovrdflg
      link override Signal_Override/_ovrdval: Value=KOUTP_LFWheelDebug_flg_ovrdval
  VTPM_LFWheelPSW_raw8_Inproc : FVT_lib/outp/OverrideAndLimit  SystemSampleTime=-1  VariantActivationTime=update diagram  Latency=0  AutoFrameSizeCalculation=off
      link override Signal_Limit/_maxval: Value=KOUTP_LFWheelPSW_raw8_maxval
      link override Signal_Limit/_minval: Value=KOUTP_LFWheelPSW_raw8_minval
      link override Signal_Override/_ovrdflg: Value=KOUTP_LFWheelPSW_raw8_ovrdflg
      link override Signal_Override/_ovrdval: Value=KOUTP_LFWheelPSW_raw8_ovrdval
  VTPM_LFWheelPress_raw8_Inproc : FVT_lib/outp/OverrideAndLimit  SystemSampleTime=-1  VariantActivationTime=update diagram  Latency=0  AutoFrameSizeCalculation=off
      link override Signal_Limit/_maxval: Value=KOUTP_LFWheelPress_raw8_maxval
      link override Signal_Limit/_minval: Value=KOUTP_LFWheelPress_raw8_minval
      link override Signal_Override/_ovrdflg: Value=KOUTP_LFWheelPress_raw8_ovrdflg
      link override Signal_Override/_ovrdval: Value=KOUTP_LFWheelPress_raw8_ovrdval
  VTPM_LFWheelTemp_C_Inproc : FVT_lib/outp/OverrideAndLimit  SystemSampleTime=-1  VariantActivationTime=update diagram  Latency=0  AutoFrameSizeCalculation=off
      link override Signal_Limit/_maxval: Value=KOUTP_LFWheelTemp_C_maxval
      link override Signal_Limit/_minval: Value=KOUTP_LFWheelTemp_C_minval
      link override Signal_Override/_ovrdflg: Value=KOUTP_LFWheelTemp_C_ovrdflg
      link override Signal_Override/_ovrdval: Value=KOUTP_LFWheelTemp_C_ovrdval
  VTPM_LFWheelTmpIndi_flg_Inproc : FVT_lib/outp/OverrideAndLimit  SystemSampleTime=-1  VariantActivationTime=update diagram  Latency=0  AutoFrameSizeCalculation=off
      link override Signal_Limit/_maxval: Value=KOUTP_LFWheelTmpIndi_flg_maxval
      link override Signal_Limit/_minval: Value=KOUTP_LFWheelTmpIndi_flg_minval
      link override Signal_Override/_ovrdflg: Value=KOUTP_LFWheelTmpIndi_flg_ovrdflg
      link override Signal_Override/_ovrdval: Value=KOUTP_LFWheelTmpIndi_flg_ovrdval
  VTPM_LRBatWarn_flg_Inproc : FVT_lib/outp/OverrideAndLimit  SystemSampleTime=-1  VariantActivationTime=update diagram  Latency=0  AutoFrameSizeCalculation=off
      link override Signal_Limit/_maxval: Value=KOUTP_LRBatWarn_flg_maxval
      link override Signal_Limit/_minval: Value=KOUTP_LRBatWarn_flg_minval
      link override Signal_Override/_ovrdflg: Value=KOUTP_LRBatWarn_flg_ovrdflg
      link override Signal_Override/_ovrdval: Value=KOUTP_LRBatWarn_flg_ovrdval
  VTPM_LRP20_raw8_Inproc : FVT_lib/outp/OverrideAndLimit  SystemSampleTime=-1  VariantActivationTime=update diagram  Latency=0  AutoFrameSizeCalculation=off
      link override Signal_Limit/_maxval: Value=KOUTP_LRP20_raw8_maxval
      link override Signal_Limit/_minval: Value=KOUTP_LRP20_raw8_minval
      link override Signal_Override/_ovrdflg: Value=KOUTP_LRP20_raw8_ovrdflg
      link override Signal_Override/_ovrdval: Value=KOUTP_LRP20_raw8_ovrdval
  VTPM_LRPindi_enum_Inproc : FVT_lib/outp/OverrideAndLimit  SystemSampleTime=-1  VariantActivationTime=update diagram  Latency=0  AutoFrameSizeCalculation=off
      link override Signal_Limit/_maxval: Value=KOUTP_LRPindi_enum_maxval
      link override Signal_Limit/_minval: Value=KOUTP_LRPindi_enum_minval
      link override Signal_Override/_ovrdflg: Value=KOUTP_LRPindi_enum_ovrdflg
      link override Signal_Override/_ovrdval: Value=KOUTP_LRPindi_enum_ovrdval
  VTPM_LRPressIndi_enum_Inproc : FVT_lib/outp/OverrideAndLimit  SystemSampleTime=-1  VariantActivationTime=update diagram  Latency=0  AutoFrameSizeCalculation=off
      link override Signal_Limit/_maxval: Value=KOUTP_LRPressIndi_enum_maxval
      link override Signal_Limit/_minval: Value=KOUTP_LRPressIndi_enum_minval
      link override Signal_Override/_ovrdflg: Value=KOUTP_LRPressIndi_enum_ovrdflg
      link override Signal_Override/_ovrdval: Value=KOUTP_LRPressIndi_enum_ovrdval
  VTPM_LRSensorFail_flg_Inproc : FVT_lib/outp/OverrideAndLimit  SystemSampleTime=-1  VariantActivationTime=update diagram  Latency=0  AutoFrameSizeCalculation=off
      link override Signal_Limit/_maxval: Value=KOUTP_LRSensorFail_flg_maxval
      link override Signal_Limit/_minval: Value=KOUTP_LRSensorFail_flg_minval
      link override Signal_Override/_ovrdflg: Value=KOUTP_LRSensorFail_flg_ovrdflg
      link override Signal_Override/_ovrdval: Value=KOUTP_LRSensorFail_flg_ovrdval
  VTPM_LRSensorMode_flg_Inproc : FVT_lib/outp/OverrideAndLimit  SystemSampleTime=-1  VariantActivationTime=update diagram  Latency=0  AutoFrameSizeCalculation=off
      link override Signal_Limit/_maxval: Value=KOUTP_LRSensorMode_flg_maxval
      link override Signal_Limit/_minval: Value=KOUTP_LRSensorMode_flg_minval
      link override Signal_Override/_ovrdflg: Value=KOUTP_LRSensorMode_flg_ovrdflg
      link override Signal_Override/_ovrdval: Value=KOUTP_LRSensorMode_flg_ovrdval
  VTPM_LRWheelDebug_flg_Inproc : FVT_lib/outp/OverrideAndLimit  SystemSampleTime=-1  VariantActivationTime=update diagram  Latency=0  AutoFrameSizeCalculation=off
      link override Signal_Limit/_maxval: Value=KOUTP_LRWheelDebug_flg_maxval
      link override Signal_Limit/_minval: Value=KOUTP_LRWheelDebug_flg_minval
      link override Signal_Override/_ovrdflg: Value=KOUTP_LRWheelDebug_flg_ovrdflg
      link override Signal_Override/_ovrdval: Value=KOUTP_LRWheelDebug_flg_ovrdval
  VTPM_LRWheelPSW_raw8_Inproc : FVT_lib/outp/OverrideAndLimit  SystemSampleTime=-1  VariantActivationTime=update diagram  Latency=0  AutoFrameSizeCalculation=off
      link override Signal_Limit/_maxval: Value=KOUTP_LRWheelPSW_raw8_maxval
      link override Signal_Limit/_minval: Value=KOUTP_LRWheelPSW_raw8_minval
      link override Signal_Override/_ovrdflg: Value=KOUTP_LRWheelPSW_raw8_ovrdflg
      link override Signal_Override/_ovrdval: Value=KOUTP_LRWheelPSW_raw8_ovrdval
  VTPM_LRWheelPress_raw8_Inproc : FVT_lib/outp/OverrideAndLimit  SystemSampleTime=-1  VariantActivationTime=update diagram  Latency=0  AutoFrameSizeCalculation=off
      link override Signal_Limit/_maxval: Value=KOUTP_LRWheelPress_raw8_maxval
      link override Signal_Limit/_minval: Value=KOUTP_LRWheelPress_raw8_minval
      link override Signal_Override/_ovrdflg: Value=KOUTP_LRWheelPress_raw8_ovrdflg
      link override Signal_Override/_ovrdval: Value=KOUTP_LRWheelPress_raw8_ovrdval
  VTPM_LRWheelTemp_C_Inproc : FVT_lib/outp/OverrideAndLimit  SystemSampleTime=-1  VariantActivationTime=update diagram  Latency=0  AutoFrameSizeCalculation=off
      link override Signal_Limit/_maxval: Value=KOUTP_LRWheelTemp_C_maxval
      link override Signal_Limit/_minval: Value=KOUTP_LRWheelTemp_C_minval
      link override Signal_Override/_ovrdflg: Value=KOUTP_LRWheelTemp_C_ovrdflg
      link override Signal_Override/_ovrdval: Value=KOUTP_LRWheelTemp_C_ovrdval
  VTPM_LRWheelTmpIndi_flg_Inproc : FVT_lib/outp/OverrideAndLimit  SystemSampleTime=-1  VariantActivationTime=update diagram  Latency=0  AutoFrameSizeCalculation=off
      link override Signal_Limit/_maxval: Value=KOUTP_LRWheelTmpIndi_flg_maxval
      link override Signal_Limit/_minval: Value=KOUTP_LRWheelTmpIndi_flg_minval
      link override Signal_Override/_ovrdflg: Value=KOUTP_LRWheelTmpIndi_flg_ovrdflg
      link override Signal_Override/_ovrdval: Value=KOUTP_LRWheelTmpIndi_flg_ovrdval
  VTPM_Prepresstempvalid_enum_Inproc : FVT_lib/outp/OverrideAndLimit  SystemSampleTime=-1  VariantActivationTime=update diagram  Latency=0  AutoFrameSizeCalculation=off
      link override Signal_Limit/_maxval: Value=KOUTP_Prepresstempvalid_enum_maxval
      link override Signal_Limit/_minval: Value=KOUTP_Prepresstempvalid_enum_minval
      link override Signal_Override/_ovrdflg: Value=KOUTP_Prepresstempvalid_enum_ovrdflg
      link override Signal_Override/_ovrdval: Value=KOUTP_Prepresstempvalid_enum_ovrdval
  VTPM_RFBatWarn_flg_Inproc : FVT_lib/outp/OverrideAndLimit  SystemSampleTime=-1  VariantActivationTime=update diagram  Latency=0  AutoFrameSizeCalculation=off
      link override Signal_Limit/_maxval: Value=KOUTP_RFBatWarn_flg_maxval
      link override Signal_Limit/_minval: Value=KOUTP_RFBatWarn_flg_minval
      link override Signal_Override/_ovrdflg: Value=KOUTP_RFBatWarn_flg_ovrdflg
      link override Signal_Override/_ovrdval: Value=KOUTP_RFBatWarn_flg_ovrdval
  VTPM_RFP20_raw8_Inproc : FVT_lib/outp/OverrideAndLimit  SystemSampleTime=-1  VariantActivationTime=update diagram  Latency=0  AutoFrameSizeCalculation=off
      link override Signal_Limit/_maxval: Value=KOUTP_RFP20_raw8_maxval
      link override Signal_Limit/_minval: Value=KOUTP_RFP20_raw8_minval
      link override Signal_Override/_ovrdflg: Value=KOUTP_RFP20_raw8_ovrdflg
      link override Signal_Override/_ovrdval: Value=KOUTP_RFP20_raw8_ovrdval
  VTPM_RFPind_enum_Inproc : FVT_lib/outp/OverrideAndLimit  SystemSampleTime=-1  VariantActivationTime=update diagram  Latency=0  AutoFrameSizeCalculation=off
      link override Signal_Limit/_maxval: Value=KOUTP_RFPind_enum_maxval
      link override Signal_Limit/_minval: Value=KOUTP_RFPind_enum_minval
      link override Signal_Override/_ovrdflg: Value=KOUTP_RFPind_enum_ovrdflg
      link override Signal_Override/_ovrdval: Value=KOUTP_RFPind_enum_ovrdval
  VTPM_RFPressIndi_enum_Inproc : FVT_lib/outp/OverrideAndLimit  SystemSampleTime=-1  VariantActivationTime=update diagram  Latency=0  AutoFrameSizeCalculation=off
      link override Signal_Limit/_maxval: Value=KOUTP_RFPressIndi_enum_maxval
      link override Signal_Limit/_minval: Value=KOUTP_RFPressIndi_enum_minval
      link override Signal_Override/_ovrdflg: Value=KOUTP_RFPressIndi_enum_ovrdflg
      link override Signal_Override/_ovrdval: Value=KOUTP_RFPressIndi_enum_ovrdval
  VTPM_RFSensorFail_flg_Inproc : FVT_lib/outp/OverrideAndLimit  SystemSampleTime=-1  VariantActivationTime=update diagram  Latency=0  AutoFrameSizeCalculation=off
      link override Signal_Limit/_maxval: Value=KOUTP_RFSensorFail_flg_maxval
      link override Signal_Limit/_minval: Value=KOUTP_RFSensorFail_flg_minval
      link override Signal_Override/_ovrdflg: Value=KOUTP_RFSensorFail_flg_ovrdflg
      link override Signal_Override/_ovrdval: Value=KOUTP_RFSensorFail_flg_ovrdval
  VTPM_RFSensorMode_flg_Inproc : FVT_lib/outp/OverrideAndLimit  SystemSampleTime=-1  VariantActivationTime=update diagram  Latency=0  AutoFrameSizeCalculation=off
      link override Signal_Limit/_maxval: Value=KOUTP_RFSensorMode_flg_maxval
      link override Signal_Limit/_minval: Value=KOUTP_RFSensorMode_flg_minval
      link override Signal_Override/_ovrdflg: Value=KOUTP_RFSensorMode_flg_ovrdflg
      link override Signal_Override/_ovrdval: Value=KOUTP_RFSensorMode_flg_ovrdval
  VTPM_RFWheelDebug_flg_Inproc : FVT_lib/outp/OverrideAndLimit  SystemSampleTime=-1  VariantActivationTime=update diagram  Latency=0  AutoFrameSizeCalculation=off
      link override Signal_Limit/_maxval: Value=KOUTP_RFWheelDebug_flg_maxval
      link override Signal_Limit/_minval: Value=KOUTP_RFWheelDebug_flg_minval
      link override Signal_Override/_ovrdflg: Value=KOUTP_RFWheelDebug_flg_ovrdflg
      link override Signal_Override/_ovrdval: Value=KOUTP_RFWheelDebug_flg_ovrdval
  VTPM_RFWheelPSW_raw8_Inproc : FVT_lib/outp/OverrideAndLimit  SystemSampleTime=-1  VariantActivationTime=update diagram  Latency=0  AutoFrameSizeCalculation=off
      link override Signal_Limit/_maxval: Value=KOUTP_RFWheelPSW_raw8_maxval
      link override Signal_Limit/_minval: Value=KOUTP_RFWheelPSW_raw8_minval
      link override Signal_Override/_ovrdflg: Value=KOUTP_RFWheelPSW_raw8_ovrdflg
      link override Signal_Override/_ovrdval: Value=KOUTP_RFWheelPSW_raw8_ovrdval
  VTPM_RFWheelPress_raw8_Inproc : FVT_lib/outp/OverrideAndLimit  SystemSampleTime=-1  VariantActivationTime=update diagram  Latency=0  AutoFrameSizeCalculation=off
      link override Signal_Limit/_maxval: Value=KOUTP_RFWheelPress_raw8_maxval
      link override Signal_Limit/_minval: Value=KOUTP_RFWheelPress_raw8_minval
      link override Signal_Override/_ovrdflg: Value=KOUTP_RFWheelPress_raw8_ovrdflg
      link override Signal_Override/_ovrdval: Value=KOUTP_RFWheelPress_raw8_ovrdval
  VTPM_RFWheelTemp_C_Inproc : FVT_lib/outp/OverrideAndLimit  SystemSampleTime=-1  VariantActivationTime=update diagram  Latency=0  AutoFrameSizeCalculation=off
      link override Signal_Limit/_maxval: Value=KOUTP_RFWheelTemp_C_maxval
      link override Signal_Limit/_minval: Value=KOUTP_RFWheelTemp_C_minval
      link override Signal_Override/_ovrdflg: Value=KOUTP_RFWheelTemp_C_ovrdflg
      link override Signal_Override/_ovrdval: Value=KOUTP_RFWheelTemp_C_ovrdval
  VTPM_RFWheelTmpIndi_flg_Inproc : FVT_lib/outp/OverrideAndLimit  SystemSampleTime=-1  VariantActivationTime=update diagram  Latency=0  AutoFrameSizeCalculation=off
      link override Signal_Limit/_maxval: Value=KOUTP_RFWheelTmpIndi_flg_maxval
      link override Signal_Limit/_minval: Value=KOUTP_RFWheelTmpIndi_flg_minval
      link override Signal_Override/_ovrdflg: Value=KOUTP_RFWheelTmpIndi_flg_ovrdflg
      link override Signal_Override/_ovrdval: Value=KOUTP_RFWheelTmpIndi_flg_ovrdval
  VTPM_RRBatWarn_flg_Inproc : FVT_lib/outp/OverrideAndLimit  SystemSampleTime=-1  VariantActivationTime=update diagram  Latency=0  AutoFrameSizeCalculation=off
      link override Signal_Limit/_maxval: Value=KOUTP_RRBatWarn_flg_maxval
      link override Signal_Limit/_minval: Value=KOUTP_RRBatWarn_flg_minval
      link override Signal_Override/_ovrdflg: Value=KOUTP_RRBatWarn_flg_ovrdflg
      link override Signal_Override/_ovrdval: Value=KOUTP_RRBatWarn_flg_ovrdval
  VTPM_RRP20_raw8_Inproc : FVT_lib/outp/OverrideAndLimit  SystemSampleTime=-1  VariantActivationTime=update diagram  Latency=0  AutoFrameSizeCalculation=off
      link override Signal_Limit/_maxval: Value=KOUTP_RRP20_raw8_maxval
      link override Signal_Limit/_minval: Value=KOUTP_RRP20_raw8_minval
      link override Signal_Override/_ovrdflg: Value=KOUTP_RRP20_raw8_ovrdflg
      link override Signal_Override/_ovrdval: Value=KOUTP_RRP20_raw8_ovrdval
  VTPM_RRPindi_enum_Inproc : FVT_lib/outp/OverrideAndLimit  SystemSampleTime=-1  VariantActivationTime=update diagram  Latency=0  AutoFrameSizeCalculation=off
      link override Signal_Limit/_maxval: Value=KOUTP_RRPindi_enum_maxval
      link override Signal_Limit/_minval: Value=KOUTP_RRPindi_enum_minval
      link override Signal_Override/_ovrdflg: Value=KOUTP_RRPindi_enum_ovrdflg
      link override Signal_Override/_ovrdval: Value=KOUTP_RRPindi_enum_ovrdval
  VTPM_RRPressIndi_enum_Inproc : FVT_lib/outp/OverrideAndLimit  SystemSampleTime=-1  VariantActivationTime=update diagram  Latency=0  AutoFrameSizeCalculation=off
      link override Signal_Limit/_maxval: Value=KOUTP_RRPressIndi_enum_maxval
      link override Signal_Limit/_minval: Value=KOUTP_RRPressIndi_enum_minval
      link override Signal_Override/_ovrdflg: Value=KOUTP_RRPressIndi_enum_ovrdflg
      link override Signal_Override/_ovrdval: Value=KOUTP_RRPressIndi_enum_ovrdval
  VTPM_RRSensorFail_flg_Inproc : FVT_lib/outp/OverrideAndLimit  SystemSampleTime=-1  VariantActivationTime=update diagram  Latency=0  AutoFrameSizeCalculation=off
      link override Signal_Limit/_maxval: Value=KOUTP_RRSensorFail_flg_maxval
      link override Signal_Limit/_minval: Value=KOUTP_RRSensorFail_flg_minval
      link override Signal_Override/_ovrdflg: Value=KOUTP_RRSensorFail_flg_ovrdflg
      link override Signal_Override/_ovrdval: Value=KOUTP_RRSensorFail_flg_ovrdval
  VTPM_RRSensorMode_flg_Inproc : FVT_lib/outp/OverrideAndLimit  SystemSampleTime=-1  VariantActivationTime=update diagram  Latency=0  AutoFrameSizeCalculation=off
      link override Signal_Limit/_maxval: Value=KOUTP_RRSensorMode_flg_maxval
      link override Signal_Limit/_minval: Value=KOUTP_RRSensorMode_flg_minval
      link override Signal_Override/_ovrdflg: Value=KOUTP_RRSensorMode_flg_ovrdflg
      link override Signal_Override/_ovrdval: Value=KOUTP_RRSensorMode_flg_ovrdval
  VTPM_RRWheelDebug_flg_Inproc : FVT_lib/outp/OverrideAndLimit  SystemSampleTime=-1  VariantActivationTime=update diagram  Latency=0  AutoFrameSizeCalculation=off
      link override Signal_Limit/_maxval: Value=KOUTP_RRWheelDebug_flg_maxval
      link override Signal_Limit/_minval: Value=KOUTP_RRWheelDebug_flg_minval
      link override Signal_Override/_ovrdflg: Value=KOUTP_RRWheelDebug_flg_ovrdflg
      link override Signal_Override/_ovrdval: Value=KOUTP_RRWheelDebug_flg_ovrdval
  VTPM_RRWheelPSW_raw8_Inproc : FVT_lib/outp/OverrideAndLimit  SystemSampleTime=-1  VariantActivationTime=update diagram  Latency=0  AutoFrameSizeCalculation=off
      link override Signal_Limit/_maxval: Value=KOUTP_RRWheelPSW_raw8_maxval
      link override Signal_Limit/_minval: Value=KOUTP_RRWheelPSW_raw8_minval
      link override Signal_Override/_ovrdflg: Value=KOUTP_RRWheelPSW_raw8_ovrdflg
      link override Signal_Override/_ovrdval: Value=KOUTP_RRWheelPSW_raw8_ovrdval
  VTPM_RRWheelPress_raw8_Inproc : FVT_lib/outp/OverrideAndLimit  SystemSampleTime=-1  VariantActivationTime=update diagram  Latency=0  AutoFrameSizeCalculation=off
      link override Signal_Limit/_maxval: Value=KOUTP_RRWheelPress_raw8_maxval
      link override Signal_Limit/_minval: Value=KOUTP_RRWheelPress_raw8_minval
      link override Signal_Override/_ovrdflg: Value=KOUTP_RRWheelPress_raw8_ovrdflg
      link override Signal_Override/_ovrdval: Value=KOUTP_RRWheelPress_raw8_ovrdval
  VTPM_RRWheelTemp_C_Inproc : FVT_lib/outp/OverrideAndLimit  SystemSampleTime=-1  VariantActivationTime=update diagram  Latency=0  AutoFrameSizeCalculation=off
      link override Signal_Limit/_maxval: Value=KOUTP_RRWheelTemp_C_maxval
      link override Signal_Limit/_minval: Value=KOUTP_RRWheelTemp_C_minval
      link override Signal_Override/_ovrdflg: Value=KOUTP_RRWheelTemp_C_ovrdflg
      link override Signal_Override/_ovrdval: Value=KOUTP_RRWheelTemp_C_ovrdval
  VTPM_RRWheelTmpIndi_flg_Inproc : FVT_lib/outp/OverrideAndLimit  SystemSampleTime=-1  VariantActivationTime=update diagram  Latency=0  AutoFrameSizeCalculation=off
      link override Signal_Limit/_maxval: Value=KOUTP_RRWheelTmpIndi_flg_maxval
      link override Signal_Limit/_minval: Value=KOUTP_RRWheelTmpIndi_flg_minval
      link override Signal_Override/_ovrdflg: Value=KOUTP_RRWheelTmpIndi_flg_ovrdflg
      link override Signal_Override/_ovrdval: Value=KOUTP_RRWheelTmpIndi_flg_ovrdval
  VTPM_S1ID_raw32_Inproc : FVT_lib/outp/OverrideAndLimit  SystemSampleTime=-1  VariantActivationTime=update diagram  Latency=0  AutoFrameSizeCalculation=off
      link override Signal_Limit/_maxval: Value=KOUTP_S1ID_raw32_maxval
      link override Signal_Limit/_minval: Value=KOUTP_S1ID_raw32_minval
      link override Signal_Override/_ovrdflg: Value=KOUTP_S1ID_raw32_ovrdflg
      link override Signal_Override/_ovrdval: Value=KOUTP_S1ID_raw32_ovrdval
  VTPM_S1L_enum_Inproc : FVT_lib/outp/OverrideAndLimit  SystemSampleTime=-1  VariantActivationTime=update diagram  Latency=0  AutoFrameSizeCalculation=off
      link override Signal_Limit/_maxval: Value=KOUTP_S1L_enum_maxval
      link override Signal_Limit/_minval: Value=KOUTP_S1L_enum_minval
      link override Signal_Override/_ovrdflg: Value=KOUTP_S1L_enum_ovrdflg
      link override Signal_Override/_ovrdval: Value=KOUTP_S1L_enum_ovrdval
  VTPM_S1WheelDebugALTU_pct_Inproc : FVT_lib/outp/OverrideAndLimit  SystemSampleTime=-1  VariantActivationTime=update diagram  Latency=0  AutoFrameSizeCalculation=off
      link override Signal_Limit/_maxval: Value=KOUTP_S1WheelDebugALTU_pct_maxval
      link override Signal_Limit/_minval: Value=KOUTP_S1WheelDebugALTU_pct_minval
      link override Signal_Override/_ovrdflg: Value=KOUTP_S1WheelDebugALTU_pct_ovrdflg
      link override Signal_Override/_ovrdval: Value=KOUTP_S1WheelDebugALTU_pct_ovrdval
  VTPM_S2ID_raw32_Inproc : FVT_lib/outp/OverrideAndLimit  SystemSampleTime=-1  VariantActivationTime=update diagram  Latency=0  AutoFrameSizeCalculation=off
      link override Signal_Limit/_maxval: Value=KOUTP_S2ID_raw32_maxval
      link override Signal_Limit/_minval: Value=KOUTP_S2ID_raw32_minval
      link override Signal_Override/_ovrdflg: Value=KOUTP_S2ID_raw32_ovrdflg
      link override Signal_Override/_ovrdval: Value=KOUTP_S2ID_raw32_ovrdval
  VTPM_S2L_enum_Inproc : FVT_lib/outp/OverrideAndLimit  SystemSampleTime=-1  VariantActivationTime=update diagram  Latency=0  AutoFrameSizeCalculation=off
      link override Signal_Limit/_maxval: Value=KOUTP_S2L_enum_maxval
      link override Signal_Limit/_minval: Value=KOUTP_S2L_enum_minval
      link override Signal_Override/_ovrdflg: Value=KOUTP_S2L_enum_ovrdflg
      link override Signal_Override/_ovrdval: Value=KOUTP_S2L_enum_ovrdval
  VTPM_S2WheelDebugALTU_pct_Inproc : FVT_lib/outp/OverrideAndLimit  SystemSampleTime=-1  VariantActivationTime=update diagram  Latency=0  AutoFrameSizeCalculation=off
      link override Signal_Limit/_maxval: Value=KOUTP_S2WheelDebugALTU_pct_maxval
      link override Signal_Limit/_minval: Value=KOUTP_S2WheelDebugALTU_pct_minval
      link override Signal_Override/_ovrdflg: Value=KOUTP_S2WheelDebugALTU_pct_ovrdflg
      link override Signal_Override/_ovrdval: Value=KOUTP_S2WheelDebugALTU_pct_ovrdval
  VTPM_S3ID_raw32_Inproc : FVT_lib/outp/OverrideAndLimit  SystemSampleTime=-1  VariantActivationTime=update diagram  Latency=0  AutoFrameSizeCalculation=off
      link override Signal_Limit/_maxval: Value=KOUTP_S3ID_raw32_maxval
      link override Signal_Limit/_minval: Value=KOUTP_S3ID_raw32_minval
      link override Signal_Override/_ovrdflg: Value=KOUTP_S3ID_raw32_ovrdflg
      link override Signal_Override/_ovrdval: Value=KOUTP_S3ID_raw32_ovrdval
  VTPM_S3L_enum_Inproc : FVT_lib/outp/OverrideAndLimit  SystemSampleTime=-1  VariantActivationTime=update diagram  Latency=0  AutoFrameSizeCalculation=off
      link override Signal_Limit/_maxval: Value=KOUTP_S3L_enum_maxval
      link override Signal_Limit/_minval: Value=KOUTP_S3L_enum_minval
      link override Signal_Override/_ovrdflg: Value=KOUTP_S3L_enum_ovrdflg
      link override Signal_Override/_ovrdval: Value=KOUTP_S3L_enum_ovrdval
  VTPM_S3WheelDebugALTU_pct_Inproc : FVT_lib/outp/OverrideAndLimit  SystemSampleTime=-1  VariantActivationTime=update diagram  Latency=0  AutoFrameSizeCalculation=off
      link override Signal_Limit/_maxval: Value=KOUTP_S3WheelDebugALTU_pct_maxval
      link override Signal_Limit/_minval: Value=KOUTP_S3WheelDebugALTU_pct_minval
      link override Signal_Override/_ovrdflg: Value=KOUTP_S3WheelDebugALTU_pct_ovrdflg
      link override Signal_Override/_ovrdval: Value=KOUTP_S3WheelDebugALTU_pct_ovrdval
  VTPM_S4ID_raw32_Inproc : FVT_lib/outp/OverrideAndLimit  SystemSampleTime=-1  VariantActivationTime=update diagram  Latency=0  AutoFrameSizeCalculation=off
      link override Signal_Limit/_maxval: Value=KOUTP_S4ID_raw32_maxval
      link override Signal_Limit/_minval: Value=KOUTP_S4ID_raw32_minval
      link override Signal_Override/_ovrdflg: Value=KOUTP_S4ID_raw32_ovrdflg
      link override Signal_Override/_ovrdval: Value=KOUTP_S4ID_raw32_ovrdval
  VTPM_S4L_enum_Inproc : FVT_lib/outp/OverrideAndLimit  SystemSampleTime=-1  VariantActivationTime=update diagram  Latency=0  AutoFrameSizeCalculation=off
      link override Signal_Limit/_maxval: Value=KOUTP_S4L_enum_maxval
      link override Signal_Limit/_minval: Value=KOUTP_S4L_enum_minval
      link override Signal_Override/_ovrdflg: Value=KOUTP_S4L_enum_ovrdflg
      link override Signal_Override/_ovrdval: Value=KOUTP_S4L_enum_ovrdval
  VTPM_S4WheelDebugALTU_pct_Inproc : FVT_lib/outp/OverrideAndLimit  SystemSampleTime=-1  VariantActivationTime=update diagram  Latency=0  AutoFrameSizeCalculation=off
      link override Signal_Limit/_maxval: Value=KOUTP_S4WheelDebugALTU_pct_maxval
      link override Signal_Limit/_minval: Value=KOUTP_S4WheelDebugALTU_pct_minval
      link override Signal_Override/_ovrdflg: Value=KOUTP_S4WheelDebugALTU_pct_ovrdflg
      link override Signal_Override/_ovrdval: Value=KOUTP_S4WheelDebugALTU_pct_ovrdval
  VTPM_SetIDLoc_flg_Inproc : FVT_lib/outp/OverrideAndLimit  SystemSampleTime=-1  VariantActivationTime=update diagram  Latency=0  AutoFrameSizeCalculation=off
      link override Signal_Limit/_maxval: Value=KOUTP_SetIDLoc_flg_maxval
      link override Signal_Limit/_minval: Value=KOUTP_SetIDLoc_flg_minval
      link override Signal_Override/_ovrdflg: Value=KOUTP_SetIDLoc_flg_ovrdflg
      link override Signal_Override/_ovrdval: Value=KOUTP_SetIDLoc_flg_ovrdval
  VTPM_TPMSCaliButtAllow_flg_Inproc : FVT_lib/outp/OverrideAndLimit  SystemSampleTime=-1  VariantActivationTime=update diagram  Latency=0  AutoFrameSizeCalculation=off
      link override Signal_Limit/_maxval: Value=KOUTP_TPMSCaliButtAllow_flg_maxval
      link override Signal_Limit/_minval: Value=KOUTP_TPMSCaliButtAllow_flg_minval
      link override Signal_Override/_ovrdflg: Value=KOUTP_TPMSCaliButtAllow_flg_ovrdflg
      link override Signal_Override/_ovrdval: Value=KOUTP_TPMSCaliButtAllow_flg_ovrdval
  VTPM_TPMSResButtAllow_flg_Inproc : FVT_lib/outp/OverrideAndLimit  SystemSampleTime=-1  VariantActivationTime=update diagram  Latency=0  AutoFrameSizeCalculation=off
      link override Signal_Limit/_maxval: Value=KOUTP_TPMSResButtAllow_flg_maxval
      link override Signal_Limit/_minval: Value=KOUTP_TPMSResButtAllow_flg_minval
      link override Signal_Override/_ovrdflg: Value=KOUTP_TPMSResButtAllow_flg_ovrdflg
      link override Signal_Override/_ovrdval: Value=KOUTP_TPMSResButtAllow_flg_ovrdval
  VTPM_TPMSResButt_flg_Inproc : FVT_lib/outp/OverrideAndLimit  SystemSampleTime=-1  VariantActivationTime=update diagram  Latency=0  AutoFrameSizeCalculation=off
      link override Signal_Limit/_maxval: Value=KOUTP_TPMSResButt_flg_maxval
      link override Signal_Limit/_minval: Value=KOUTP_TPMSResButt_flg_minval
      link override Signal_Override/_ovrdflg: Value=KOUTP_TPMSResButt_flg_ovrdflg
      link override Signal_Override/_ovrdval: Value=KOUTP_TPMSResButt_flg_ovrdval
  VTPM_TPMSStorge_flg_Inproc : FVT_lib/outp/OverrideAndLimit  SystemSampleTime=-1  VariantActivationTime=update diagram  Latency=0  AutoFrameSizeCalculation=off
      link override Signal_Limit/_maxval: Value=KOUTP_TPMSStorge_flg_maxval
      link override Signal_Limit/_minval: Value=KOUTP_TPMSStorge_flg_minval
      link override Signal_Override/_ovrdflg: Value=KOUTP_TPMSStorge_flg_ovrdflg
      link override Signal_Override/_ovrdval: Value=KOUTP_TPMSStorge_flg_ovrdval
  VTPM_TPMSWarnIndi_enum_Inproc : FVT_lib/outp/OverrideAndLimit  SystemSampleTime=-1  VariantActivationTime=update diagram  Latency=0  AutoFrameSizeCalculation=off
      link override Signal_Limit/_maxval: Value=KOUTP_TPMSWarnIndi_enum_maxval
      link override Signal_Limit/_minval: Value=KOUTP_TPMSWarnIndi_enum_minval
      link override Signal_Override/_ovrdflg: Value=KOUTP_TPMSWarnIndi_enum_ovrdflg
      link override Signal_Override/_ovrdval: Value=KOUTP_TPMSWarnIndi_enum_ovrdval
  VTPM_WriteChkLFID_raw_Inproc : FVT_lib/outp/OverrideAndLimit  SystemSampleTime=-1  VariantActivationTime=update diagram  Latency=0  AutoFrameSizeCalculation=off
      link override Signal_Limit/_maxval: Value=KOUTP_WriteChkLFID_raw_maxval
      link override Signal_Limit/_minval: Value=KOUTP_WriteChkLFID_raw_minval
      link override Signal_Override/_ovrdflg: Value=KOUTP_WriteChkLFID_raw_ovrdflg
      link override Signal_Override/_ovrdval: Value=KOUTP_WriteChkLFID_raw_ovrdval
  VTPM_WriteChkLRID_raw_Inproc : FVT_lib/outp/OverrideAndLimit  SystemSampleTime=-1  VariantActivationTime=update diagram  Latency=0  AutoFrameSizeCalculation=off
      link override Signal_Limit/_maxval: Value=KOUTP_WriteChkLRID_raw_maxval
      link override Signal_Limit/_minval: Value=KOUTP_WriteChkLRID_raw_minval
      link override Signal_Override/_ovrdflg: Value=KOUTP_WriteChkLRID_raw_ovrdflg
      link override Signal_Override/_ovrdval: Value=KOUTP_WriteChkLRID_raw_ovrdval
  VTPM_WriteChkRFID_raw_Inproc : FVT_lib/outp/OverrideAndLimit  SystemSampleTime=-1  VariantActivationTime=update diagram  Latency=0  AutoFrameSizeCalculation=off
      link override Signal_Limit/_maxval: Value=KOUTP_WriteChkRFID_raw_maxval
      link override Signal_Limit/_minval: Value=KOUTP_WriteChkRFID_raw_minval
      link override Signal_Override/_ovrdflg: Value=KOUTP_WriteChkRFID_raw_ovrdflg
      link override Signal_Override/_ovrdval: Value=KOUTP_WriteChkRFID_raw_ovrdval
  VTPM_WriteChkRRID_raw_Inproc : FVT_lib/outp/OverrideAndLimit  SystemSampleTime=-1  VariantActivationTime=update diagram  Latency=0  AutoFrameSizeCalculation=off
      link override Signal_Limit/_maxval: Value=KOUTP_WriteChkRRID_raw_maxval
      link override Signal_Limit/_minval: Value=KOUTP_WriteChkRRID_raw_minval
      link override Signal_Override/_ovrdflg: Value=KOUTP_WriteChkRRID_raw_ovrdflg
      link override Signal_Override/_ovrdval: Value=KOUTP_WriteChkRRID_raw_ovrdval
  VTPM_WriteChkfinLFID_raw_Inproc : FVT_lib/outp/OverrideAndLimit  SystemSampleTime=-1  VariantActivationTime=update diagram  Latency=0  AutoFrameSizeCalculation=off
      link override Signal_Limit/_maxval: Value=KOUTP_WriteChkfinLFID_raw_maxval
      link override Signal_Limit/_minval: Value=KOUTP_WriteChkfinLFID_raw_minval
      link override Signal_Override/_ovrdflg: Value=KOUTP_WriteChkfinLFID_raw_ovrdflg
      link override Signal_Override/_ovrdval: Value=KOUTP_WriteChkfinLFID_raw_ovrdval
  VTPM_WriteChkfinLRID_raw_Inproc : FVT_lib/outp/OverrideAndLimit  SystemSampleTime=-1  VariantActivationTime=update diagram  Latency=0  AutoFrameSizeCalculation=off
      link override Signal_Limit/_maxval: Value=KOUTP_WriteChkfinLRID_raw_maxval
      link override Signal_Limit/_minval: Value=KOUTP_WriteChkfinLRID_raw_minval
      link override Signal_Override/_ovrdflg: Value=KOUTP_WriteChkfinLRID_raw_ovrdflg
      link override Signal_Override/_ovrdval: Value=KOUTP_WriteChkfinLRID_raw_ovrdval
  VTPM_WriteChkfinRFID_raw_Inproc : FVT_lib/outp/OverrideAndLimit  SystemSampleTime=-1  VariantActivationTime=update diagram  Latency=0  AutoFrameSizeCalculation=off
      link override Signal_Limit/_maxval: Value=KOUTP_WriteChkfinRFID_raw_maxval
      link override Signal_Limit/_minval: Value=KOUTP_WriteChkfinRFID_raw_minval
      link override Signal_Override/_ovrdflg: Value=KOUTP_WriteChkfinRFID_raw_ovrdflg
      link override Signal_Override/_ovrdval: Value=KOUTP_WriteChkfinRFID_raw_ovrdval
  VTPM_WriteChkfinRRID_raw_Inproc : FVT_lib/outp/OverrideAndLimit  SystemSampleTime=-1  VariantActivationTime=update diagram  Latency=0  AutoFrameSizeCalculation=off
      link override Signal_Limit/_maxval: Value=KOUTP_WriteChkfinRRID_raw_maxval
      link override Signal_Limit/_minval: Value=KOUTP_WriteChkfinRRID_raw_minval
      link override Signal_Override/_ovrdflg: Value=KOUTP_WriteChkfinRRID_raw_ovrdflg
      link override Signal_Override/_ovrdval: Value=KOUTP_WriteChkfinRRID_raw_ovrdval
  VTPM_unlearnSfailvalid_enum_Inproc : FVT_lib/outp/OverrideAndLimit  SystemSampleTime=-1  VariantActivationTime=update diagram  Latency=0  AutoFrameSizeCalculation=off
      link override Signal_Limit/_maxval: Value=KOUTP_unlearnSfailvalid_enum_maxval
      link override Signal_Limit/_minval: Value=KOUTP_unlearnSfailvalid_enum_minval
      link override Signal_Override/_ovrdflg: Value=KOUTP_unlearnSfailvalid_enum_ovrdflg
      link override Signal_Override/_ovrdval: Value=KOUTP_unlearnSfailvalid_enum_ovrdval
  VTPM_unlearnSfali_flg_Inproc : FVT_lib/outp/OverrideAndLimit  SystemSampleTime=-1  VariantActivationTime=update diagram  Latency=0  AutoFrameSizeCalculation=off
      link override Signal_Limit/_maxval: Value=KOUTP_unlearnSfali_flg_maxval
      link override Signal_Limit/_minval: Value=KOUTP_unlearnSfali_flg_minval
      link override Signal_Override/_ovrdflg: Value=KOUTP_unlearnSfali_flg_ovrdflg
      link override Signal_Override/_ovrdval: Value=KOUTP_unlearnSfali_flg_ovrdval
  VTQD_AccPedal1LowSW_enum_Inproc : FVT_lib/outp/OverrideAndLimit  SystemSampleTime=-1  VariantActivationTime=update diagram  Latency=0  AutoFrameSizeCalculation=off
      link override Signal_Limit/_maxval: Value=KOUTP_AccPedal1LowSW_enum_maxval
      link override Signal_Limit/_minval: Value=KOUTP_AccPedal1LowSW_enum_minval
      link override Signal_Override/_ovrdflg: Value=KOUTP_AccPedal1LowSW_enum_ovrdflg
      link override Signal_Override/_ovrdval: Value=KOUTP_AccPedal1LowSW_enum_ovrdval
  VTQD_AccPedalPos1_pct_Inproc : FVT_lib/outp/OverrideAndLimit  SystemSampleTime=-1  VariantActivationTime=update diagram  Latency=0  AutoFrameSizeCalculation=off
      link override Signal_Limit/_maxval: Value=KOUTP_AccPedalPos1_pct_maxval
      link override Signal_Limit/_minval: Value=KOUTP_AccPedalPos1_pct_minval
      link override Signal_Override/_ovrdflg: Value=KOUTP_AccPedalPos1_pct_ovrdflg
      link override Signal_Override/_ovrdval: Value=KOUTP_AccPedalPos1_pct_ovrdval
  VTQD_ActDriveDirect_enum_Inproc : FVT_lib/outp/OverrideAndLimit  SystemSampleTime=-1  VariantActivationTime=update diagram  Latency=0  AutoFrameSizeCalculation=off
      link override Signal_Limit/_maxval: Value=KOUTP_ActDriveDirect_enum_maxval
      link override Signal_Limit/_minval: Value=KOUTP_ActDriveDirect_enum_minval
      link override Signal_Override/_ovrdflg: Value=KOUTP_ActDriveDirect_enum_ovrdflg
      link override Signal_Override/_ovrdval: Value=KOUTP_ActDriveDirect_enum_ovrdval
  VTQD_ActEMOutSftSpd_rpm_Inproc : FVT_lib/outp/OverrideAndLimit  SystemSampleTime=-1  VariantActivationTime=update diagram  Latency=0  AutoFrameSizeCalculation=off
      link override Signal_Limit/_maxval: Value=KOUTP_ActEMOutSftSpd_rpm_maxval
      link override Signal_Limit/_minval: Value=KOUTP_ActEMOutSftSpd_rpm_minval
      link override Signal_Override/_ovrdflg: Value=KOUTP_ActEMOutSftSpd_rpm_ovrdflg
      link override Signal_Override/_ovrdval: Value=KOUTP_ActEMOutSftSpd_rpm_ovrdval
  VTQD_ActEMpTrqHrls_pct_Inproc : FVT_lib/outp/OverrideAndLimit  SystemSampleTime=-1  VariantActivationTime=update diagram  Latency=0  AutoFrameSizeCalculation=off
      link override Signal_Limit/_maxval: Value=KOUTP_ActEMpTrqHrls_pct_maxval
      link override Signal_Limit/_minval: Value=KOUTP_ActEMpTrqHrls_pct_minval
      link override Signal_Override/_ovrdflg: Value=KOUTP_ActEMpTrqHrls_pct_ovrdflg
      link override Signal_Override/_ovrdval: Value=KOUTP_ActEMpTrqHrls_pct_ovrdval
  VTQD_ActEMpTrq_pct_Inproc : FVT_lib/outp/OverrideAndLimit  SystemSampleTime=-1  VariantActivationTime=update diagram  Latency=0  AutoFrameSizeCalculation=off
      link override Signal_Limit/_maxval: Value=KOUTP_ActEMpTrq_pct_maxval
      link override Signal_Limit/_minval: Value=KOUTP_ActEMpTrq_pct_minval
      link override Signal_Override/_ovrdflg: Value=KOUTP_ActEMpTrq_pct_ovrdflg
      link override Signal_Override/_ovrdval: Value=KOUTP_ActEMpTrq_pct_ovrdval
  VTQD_ActMaxAvaEMRecpTrq_pct_Inproc : FVT_lib/outp/OverrideAndLimit  SystemSampleTime=-1  VariantActivationTime=update diagram  Latency=0  AutoFrameSizeCalculation=off
      link override Signal_Limit/_maxval: Value=KOUTP_ActMaxAvaEMRecpTrq_pct_maxval
      link override Signal_Limit/_minval: Value=KOUTP_ActMaxAvaEMRecpTrq_pct_minval
      link override Signal_Override/_ovrdflg: Value=KOUTP_ActMaxAvaEMRecpTrq_pct_ovrdflg
      link override Signal_Override/_ovrdval: Value=KOUTP_ActMaxAvaEMRecpTrq_pct_ovrdval
  VTQD_BrakeSW_enum_Inproc : FVT_lib/outp/OverrideAndLimit  SystemSampleTime=-1  VariantActivationTime=update diagram  Latency=0  AutoFrameSizeCalculation=off
      link override Signal_Limit/_maxval: Value=KOUTP_BrakeSW_enum_maxval
      link override Signal_Limit/_minval: Value=KOUTP_BrakeSW_enum_minval
      link override Signal_Override/_ovrdflg: Value=KOUTP_BrakeSW_enum_ovrdflg
      link override Signal_Override/_ovrdval: Value=KOUTP_BrakeSW_enum_ovrdval
  VTQD_CreepON_flg_Inproc : FVT_lib/outp/OverrideAndLimit  SystemSampleTime=-1  VariantActivationTime=update diagram  Latency=0  AutoFrameSizeCalculation=off
      link override Signal_Limit/_maxval: Value=KOUTP_CreepON_flg_maxval
      link override Signal_Limit/_minval: Value=KOUTP_CreepON_flg_minval
      link override Signal_Override/_ovrdflg: Value=KOUTP_CreepON_flg_ovrdflg
      link override Signal_Override/_ovrdval: Value=KOUTP_CreepON_flg_ovrdval
  VTQD_DLEngaged_enum_Inproc : FVT_lib/outp/OverrideAndLimit  SystemSampleTime=-1  VariantActivationTime=update diagram  Latency=0  AutoFrameSizeCalculation=off
      link override Signal_Limit/_maxval: Value=KOUTP_DLEngaged_enum_maxval
      link override Signal_Limit/_minval: Value=KOUTP_DLEngaged_enum_minval
      link override Signal_Override/_ovrdflg: Value=KOUTP_DLEngaged_enum_ovrdflg
      link override Signal_Override/_ovrdval: Value=KOUTP_DLEngaged_enum_ovrdval
  VTQD_DriverWhlTqDemFr_Nm_Inproc : FVT_lib/outp/OverrideAndLimit  SystemSampleTime=-1  VariantActivationTime=update diagram  Latency=0  AutoFrameSizeCalculation=off
      link override Signal_Limit/_maxval: Value=KOUTP_DriverWhlTqDemFr_Nm_maxval
      link override Signal_Limit/_minval: Value=KOUTP_DriverWhlTqDemFr_Nm_minval
      link override Signal_Override/_ovrdflg: Value=KOUTP_DriverWhlTqDemFr_Nm_ovrdflg
      link override Signal_Override/_ovrdval: Value=KOUTP_DriverWhlTqDemFr_Nm_ovrdval
  VTQD_DriverWhlTqDemRr_Nm_Inproc : FVT_lib/outp/OverrideAndLimit  SystemSampleTime=-1  VariantActivationTime=update diagram  Latency=0  AutoFrameSizeCalculation=off
      link override Signal_Limit/_maxval: Value=KOUTP_DriverWhlTqDemRr_Nm_maxval
      link override Signal_Limit/_minval: Value=KOUTP_DriverWhlTqDemRr_Nm_minval
      link override Signal_Override/_ovrdflg: Value=KOUTP_DriverWhlTqDemRr_Nm_ovrdflg
      link override Signal_Override/_ovrdval: Value=KOUTP_DriverWhlTqDemRr_Nm_ovrdval
  VTQD_DrvDemEMRtapTrq_pct_Inproc : FVT_lib/outp/OverrideAndLimit  SystemSampleTime=-1  VariantActivationTime=update diagram  Latency=0  AutoFrameSizeCalculation=off
      link override Signal_Limit/_maxval: Value=KOUTP_DrvDemEMRtapTrq_pct_maxval
      link override Signal_Limit/_minval: Value=KOUTP_DrvDemEMRtapTrq_pct_minval
      link override Signal_Override/_ovrdflg: Value=KOUTP_DrvDemEMRtapTrq_pct_ovrdflg
      link override Signal_Override/_ovrdval: Value=KOUTP_DrvDemEMRtapTrq_pct_ovrdval
  VTQD_EEC2MSGCS_raw_Inproc : FVT_lib/outp/OverrideAndLimit  SystemSampleTime=-1  VariantActivationTime=update diagram  Latency=0  AutoFrameSizeCalculation=off
      link override Signal_Limit/_maxval: Value=KOUTP_EEC2MSGCS_raw_maxval
      link override Signal_Limit/_minval: Value=KOUTP_EEC2MSGCS_raw_minval
      link override Signal_Override/_ovrdflg: Value=KOUTP_EEC2MSGCS_raw_ovrdflg
      link override Signal_Override/_ovrdval: Value=KOUTP_EEC2MSGCS_raw_ovrdval
  VTQD_EEC2MSGCnt_raw_Inproc : FVT_lib/outp/OverrideAndLimit  SystemSampleTime=-1  VariantActivationTime=update diagram  Latency=0  AutoFrameSizeCalculation=off
      link override Signal_Limit/_maxval: Value=KOUTP_EEC2MSGCnt_raw_maxval
      link override Signal_Limit/_minval: Value=KOUTP_EEC2MSGCnt_raw_minval
      link override Signal_Override/_ovrdflg: Value=KOUTP_EEC2MSGCnt_raw_ovrdflg
      link override Signal_Override/_ovrdval: Value=KOUTP_EEC2MSGCnt_raw_ovrdval
  VTQD_EMParasLoss_pct_Inproc : FVT_lib/outp/OverrideAndLimit  SystemSampleTime=-1  VariantActivationTime=update diagram  Latency=0  AutoFrameSizeCalculation=off
      link override Signal_Limit/_maxval: Value=KOUTP_EMParasLoss_pct_maxval
      link override Signal_Limit/_minval: Value=KOUTP_EMParasLoss_pct_minval
      link override Signal_Override/_ovrdflg: Value=KOUTP_EMParasLoss_pct_ovrdflg
      link override Signal_Override/_ovrdval: Value=KOUTP_EMParasLoss_pct_ovrdval
  VTQD_EMTrqModeDrvBrk_enum_Inproc : FVT_lib/outp/OverrideAndLimit  SystemSampleTime=-1  VariantActivationTime=update diagram  Latency=0  AutoFrameSizeCalculation=off
      link override Signal_Limit/_maxval: Value=KOUTP_EMTrqModeDrvBrk_enum_maxval
      link override Signal_Limit/_minval: Value=KOUTP_EMTrqModeDrvBrk_enum_minval
      link override Signal_Override/_ovrdflg: Value=KOUTP_EMTrqModeDrvBrk_enum_ovrdflg
      link override Signal_Override/_ovrdval: Value=KOUTP_EMTrqModeDrvBrk_enum_ovrdval
  VTQD_EVDriveMode_enum_Inproc : FVT_lib/outp/OverrideAndLimit  SystemSampleTime=-1  VariantActivationTime=update diagram  Latency=0  AutoFrameSizeCalculation=off
      link override Signal_Limit/_maxval: Value=KOUTP_EVDriveMode_enum_maxval
      link override Signal_Limit/_minval: Value=KOUTP_EVDriveMode_enum_minval
      link override Signal_Override/_ovrdflg: Value=KOUTP_EVDriveMode_enum_ovrdflg
      link override Signal_Override/_ovrdval: Value=KOUTP_EVDriveMode_enum_ovrdval
  VTQD_FDCCHAEBSHBSwSta_enum_Inproc : FVT_lib/outp/OverrideAndLimit  SystemSampleTime=-1  VariantActivationTime=update diagram  Latency=0  AutoFrameSizeCalculation=off
      link override Signal_Limit/_maxval: Value=KOUTP_FDCCHAEBSHBSwSta_enum_maxval
      link override Signal_Limit/_minval: Value=KOUTP_FDCCHAEBSHBSwSta_enum_minval
      link override Signal_Override/_ovrdflg: Value=KOUTP_FDCCHAEBSHBSwSta_enum_ovrdflg
      link override Signal_Override/_ovrdval: Value=KOUTP_FDCCHAEBSHBSwSta_enum_ovrdval
  VTQD_FDCCHAEBSHHSwSta_enum_Inproc : FVT_lib/outp/OverrideAndLimit  SystemSampleTime=-1  VariantActivationTime=update diagram  Latency=0  AutoFrameSizeCalculation=off
      link override Signal_Limit/_maxval: Value=KOUTP_FDCCHAEBSHHSwSta_enum_maxval
      link override Signal_Limit/_minval: Value=KOUTP_FDCCHAEBSHHSwSta_enum_minval
      link override Signal_Override/_ovrdflg: Value=KOUTP_FDCCHAEBSHHSwSta_enum_ovrdflg
      link override Signal_Override/_ovrdval: Value=KOUTP_FDCCHAEBSHHSwSta_enum_ovrdval
  VTQD_FDCCHAEBSRd4BRSta_enum_Inproc : FVT_lib/outp/OverrideAndLimit  SystemSampleTime=-1  VariantActivationTime=update diagram  Latency=0  AutoFrameSizeCalculation=off
      link override Signal_Limit/_maxval: Value=KOUTP_FDCCHAEBSRd4BRSta_enum_maxval
      link override Signal_Limit/_minval: Value=KOUTP_FDCCHAEBSRd4BRSta_enum_minval
      link override Signal_Override/_ovrdflg: Value=KOUTP_FDCCHAEBSRd4BRSta_enum_ovrdflg
      link override Signal_Override/_ovrdval: Value=KOUTP_FDCCHAEBSRd4BRSta_enum_ovrdval
  VTQD_FDCVCUDACStatusSta_enum_Inproc : FVT_lib/outp/OverrideAndLimit  SystemSampleTime=-1  VariantActivationTime=update diagram  Latency=0  AutoFrameSizeCalculation=off
      link override Signal_Limit/_maxval: Value=KOUTP_FDCVCUDACStatusSta_enum_maxval
      link override Signal_Limit/_minval: Value=KOUTP_FDCVCUDACStatusSta_enum_minval
      link override Signal_Override/_ovrdflg: Value=KOUTP_FDCVCUDACStatusSta_enum_ovrdflg
      link override Signal_Override/_ovrdval: Value=KOUTP_FDCVCUDACStatusSta_enum_ovrdval
  VTQD_FDCVCUTUpAStaSta_enum_Inproc : FVT_lib/outp/OverrideAndLimit  SystemSampleTime=-1  VariantActivationTime=update diagram  Latency=0  AutoFrameSizeCalculation=off
      link override Signal_Limit/_maxval: Value=KOUTP_FDCVCUTUpAStaSta_enum_maxval
      link override Signal_Limit/_minval: Value=KOUTP_FDCVCUTUpAStaSta_enum_minval
      link override Signal_Override/_ovrdflg: Value=KOUTP_FDCVCUTUpAStaSta_enum_ovrdflg
      link override Signal_Override/_ovrdval: Value=KOUTP_FDCVCUTUpAStaSta_enum_ovrdval
  VTQD_FrActvDmpDisabReq_flg_Inproc : FVT_lib/outp/OverrideAndLimit  SystemSampleTime=-1  VariantActivationTime=update diagram  Latency=0  AutoFrameSizeCalculation=off
      link override Signal_Limit/_maxval: Value=KOUTP_FrActvDmpDisabReq_flg_maxval
      link override Signal_Limit/_minval: Value=KOUTP_FrActvDmpDisabReq_flg_minval
      link override Signal_Override/_ovrdflg: Value=KOUTP_FrActvDmpDisabReq_flg_ovrdflg
      link override Signal_Override/_ovrdval: Value=KOUTP_FrActvDmpDisabReq_flg_ovrdval
  VTQD_FrEDUActTq_Nm_Inproc : FVT_lib/outp/OverrideAndLimit  SystemSampleTime=-1  VariantActivationTime=update diagram  Latency=0  AutoFrameSizeCalculation=off
      link override Signal_Limit/_maxval: Value=KOUTP_FrEDUActTq_Nm_maxval
      link override Signal_Limit/_minval: Value=KOUTP_FrEDUActTq_Nm_minval
      link override Signal_Override/_ovrdflg: Value=KOUTP_FrEDUActTq_Nm_ovrdflg
      link override Signal_Override/_ovrdval: Value=KOUTP_FrEDUActTq_Nm_ovrdval
  VTQD_FrEDUAvailBrkRgnTqV_flg_Inproc : FVT_lib/outp/OverrideAndLimit  SystemSampleTime=-1  VariantActivationTime=update diagram  Latency=0  AutoFrameSizeCalculation=off
      link override Signal_Limit/_maxval: Value=KOUTP_FrEDUAvailBrkRgnTqV_flg_maxval
      link override Signal_Limit/_minval: Value=KOUTP_FrEDUAvailBrkRgnTqV_flg_minval
      link override Signal_Override/_ovrdflg: Value=KOUTP_FrEDUAvailBrkRgnTqV_flg_ovrdflg
      link override Signal_Override/_ovrdval: Value=KOUTP_FrEDUAvailBrkRgnTqV_flg_ovrdval
  VTQD_FrEDUAvailBrkRgnTq_Nm_Inproc : FVT_lib/outp/OverrideAndLimit  SystemSampleTime=-1  VariantActivationTime=update diagram  Latency=0  AutoFrameSizeCalculation=off
      link override Signal_Limit/_maxval: Value=KOUTP_FrEDUAvailBrkRgnTq_Nm_maxval
      link override Signal_Limit/_minval: Value=KOUTP_FrEDUAvailBrkRgnTq_Nm_minval
      link override Signal_Override/_ovrdflg: Value=KOUTP_FrEDUAvailBrkRgnTq_Nm_ovrdflg
      link override Signal_Override/_ovrdval: Value=KOUTP_FrEDUAvailBrkRgnTq_Nm_ovrdval
  VTQD_FrEDURolRgnTq_Nm_Inproc : FVT_lib/outp/OverrideAndLimit  SystemSampleTime=-1  VariantActivationTime=update diagram  Latency=0  AutoFrameSizeCalculation=off
      link override Signal_Limit/_maxval: Value=KOUTP_FrEDURolRgnTq_Nm_maxval
      link override Signal_Limit/_minval: Value=KOUTP_FrEDURolRgnTq_Nm_minval
      link override Signal_Override/_ovrdflg: Value=KOUTP_FrEDURolRgnTq_Nm_ovrdflg
      link override Signal_Override/_ovrdval: Value=KOUTP_FrEDURolRgnTq_Nm_ovrdval
  VTQD_FrEDUSpdValid_flg_Inproc : FVT_lib/outp/OverrideAndLimit  SystemSampleTime=-1  VariantActivationTime=update diagram  Latency=0  AutoFrameSizeCalculation=off
      link override Signal_Limit/_maxval: Value=KOUTP_FrEDUSpdValid_flg_maxval
      link override Signal_Limit/_minval: Value=KOUTP_FrEDUSpdValid_flg_minval
      link override Signal_Override/_ovrdflg: Value=KOUTP_FrEDUSpdValid_flg_ovrdflg
      link override Signal_Override/_ovrdval: Value=KOUTP_FrEDUSpdValid_flg_ovrdval
  VTQD_FrEDUSpd_rpm_Inproc : FVT_lib/outp/OverrideAndLimit  SystemSampleTime=-1  VariantActivationTime=update diagram  Latency=0  AutoFrameSizeCalculation=off
      link override Signal_Limit/_maxval: Value=KOUTP_FrEDUSpd_rpm_maxval
      link override Signal_Limit/_minval: Value=KOUTP_FrEDUSpd_rpm_minval
      link override Signal_Override/_ovrdflg: Value=KOUTP_FrEDUSpd_rpm_ovrdflg
      link override Signal_Override/_ovrdval: Value=KOUTP_FrEDUSpd_rpm_ovrdval
  VTQD_FrIdcMax_A_Inproc : FVT_lib/outp/OverrideAndLimit  SystemSampleTime=-1  VariantActivationTime=update diagram  Latency=0  AutoFrameSizeCalculation=off
      link override Signal_Limit/_maxval: Value=KOUTP_FrIdcMax_A_maxval
      link override Signal_Limit/_minval: Value=KOUTP_FrIdcMax_A_minval
      link override Signal_Override/_ovrdflg: Value=KOUTP_FrIdcMax_A_ovrdflg
      link override Signal_Override/_ovrdval: Value=KOUTP_FrIdcMax_A_ovrdval
  VTQD_FrIdcMin_A_Inproc : FVT_lib/outp/OverrideAndLimit  SystemSampleTime=-1  VariantActivationTime=update diagram  Latency=0  AutoFrameSizeCalculation=off
      link override Signal_Limit/_maxval: Value=KOUTP_FrIdcMin_A_maxval
      link override Signal_Limit/_minval: Value=KOUTP_FrIdcMin_A_minval
      link override Signal_Override/_ovrdflg: Value=KOUTP_FrIdcMin_A_ovrdflg
      link override Signal_Override/_ovrdval: Value=KOUTP_FrIdcMin_A_ovrdval
  VTQD_FrRgnDecrSta_flg_Inproc : FVT_lib/outp/OverrideAndLimit  SystemSampleTime=-1  VariantActivationTime=update diagram  Latency=0  AutoFrameSizeCalculation=off
      link override Signal_Limit/_maxval: Value=KOUTP_FrRgnDecrSta_flg_maxval
      link override Signal_Limit/_minval: Value=KOUTP_FrRgnDecrSta_flg_minval
      link override Signal_Override/_ovrdflg: Value=KOUTP_FrRgnDecrSta_flg_ovrdflg
      link override Signal_Override/_ovrdval: Value=KOUTP_FrRgnDecrSta_flg_ovrdval
  VTQD_FrRgnPermSta_flg_Inproc : FVT_lib/outp/OverrideAndLimit  SystemSampleTime=-1  VariantActivationTime=update diagram  Latency=0  AutoFrameSizeCalculation=off
      link override Signal_Limit/_maxval: Value=KOUTP_FrRgnPermSta_flg_maxval
      link override Signal_Limit/_minval: Value=KOUTP_FrRgnPermSta_flg_minval
      link override Signal_Override/_ovrdflg: Value=KOUTP_FrRgnPermSta_flg_ovrdflg
      link override Signal_Override/_ovrdval: Value=KOUTP_FrRgnPermSta_flg_ovrdval
  VTQD_FrUdcMax_V_Inproc : FVT_lib/outp/OverrideAndLimit  SystemSampleTime=-1  VariantActivationTime=update diagram  Latency=0  AutoFrameSizeCalculation=off
      link override Signal_Limit/_maxval: Value=KOUTP_FrUdcMax_V_maxval
      link override Signal_Limit/_minval: Value=KOUTP_FrUdcMax_V_minval
      link override Signal_Override/_ovrdflg: Value=KOUTP_FrUdcMax_V_ovrdflg
